simulink model "LF_AC29bus_HVDCdemo_V2_1"  (R2019b)
settings: Solver=FixedStepDiscrete  StartTime=0.0  StopTime=fix(6/Ts)*Ts  FixedStep=Ts  RelTol=1e-3
InitFcn:
  | Ts_avg=150e-6;
  | Ts=50e-6;
  | 
  | %Tc_stab = 1/60/5;
  | %Tc_stab = 2/60;
  | Tc_stab = Ts;
  | 
  | 
  | Ts_avg=150e-6;
  | 
  | Ts=50e-6;
  | 
  | % Rectifier AC side :
  | VLL_nom_R = 735e3; % V
  | Fnom_R = 60;           % Hz
  | 
  | % Inverter AC side :
  | VLL_nom_I = 735e3; % V
  | Fnom_I = 60;           % Hz
  | 
  | % DC :
  | Vdc_nom = 500e3;   % V
  | Idc_nom  = 2000;     % A
undefined symbols (not defined in the file): D1, D11, Delta, test_alpha
libraries: powerlib x223, powerlib_meascontrol x57, simulink x22, sps_avr x7
(part 3 of 10)

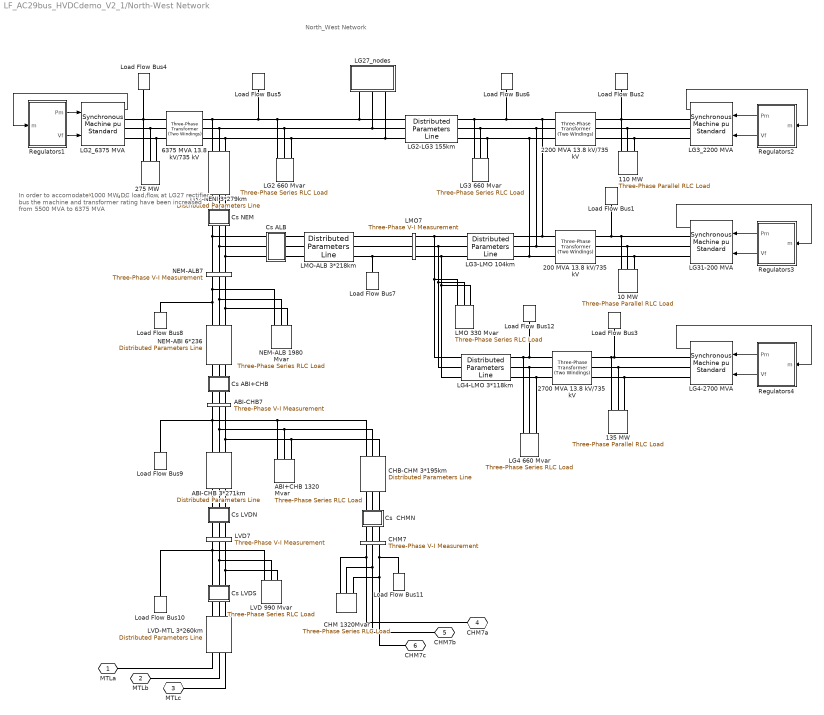
== system LF_AC29bus_HVDCdemo_V2_1/North-West Network ==
  note: North_West Network
  note: In order to accomodate 1000 MW
      | DC load flow at LG27 rectifier bus
      | the machine and transformer rating have been
      | increased from 5500 MVA to 6375 MVA
  10 MW : powerlib/Elements/Three-Phase Parallel RLC Load  LConnTagsString=A|B|C  Configuration=Y (grounded)  NominalVoltage=(13800)*1  Vabc=[1e3 1e3 1e3]  Vabcp=[1e3 1e3 1e3]  NominalFrequency=60  UnbalancedPower=off  ActivePower=10000000  InductivePower=0  CapacitivePower=0  Pabc=[10e3 9e3 11e3]  QLabc=[100 90 110]  QCabc=[100 90 110]  Pabcp=[10e3 9e3 11e3]  QLabcp=[100 90 110]  QCabcp=[100 90 110]  Measurements=None  LoadType=constant PQ
      settings: SourceProductName=Simscape Electrical
  110 MW : powerlib/Elements/Three-Phase Parallel RLC Load  LConnTagsString=A|B|C  Configuration=Y (grounded)  NominalVoltage=(13800)*1  Vabc=[1e3 1e3 1e3]  Vabcp=[1e3 1e3 1e3]  NominalFrequency=60  UnbalancedPower=off  ActivePower=110000000  InductivePower=0  CapacitivePower=0  Pabc=[10e3 9e3 11e3]  QLabc=[100 90 110]  QCabc=[100 90 110]  Pabcp=[10e3 9e3 11e3]  QLabcp=[100 90 110]  QCabcp=[100 90 110]  Measurements=None  LoadType=constant PQ
      settings: SourceProductName=Simscape Electrical
  135 MW : powerlib/Elements/Three-Phase Parallel RLC Load  LConnTagsString=A|B|C  Configuration=Y (grounded)  NominalVoltage=(13800)*1  Vabc=[1e3 1e3 1e3]  Vabcp=[1e3 1e3 1e3]  NominalFrequency=60  UnbalancedPower=off  ActivePower=135000000  InductivePower=0  CapacitivePower=0  Pabc=[10e3 9e3 11e3]  QLabc=[100 90 110]  QCabc=[100 90 110]  Pabcp=[10e3 9e3 11e3]  QLabcp=[100 90 110]  QCabcp=[100 90 110]  Measurements=None  LoadType=constant PQ
      settings: SourceProductName=Simscape Electrical
  200 MVA 13.8 kV/735 kV : powerlib/Elements/Three-Phase Transformer (Two Windings)  Winding1Connection=Delta (D1)  Winding2Connection=Yg  CoreType=Three single-phase transformers  SetSaturation=off  Hysteresis=off  DataFile='basic_model'  SetInitialFlux=off  Measurements=None  UNITS=pu  NominalPower=[ 200e6 60 ]  Winding1="[ 13.8e3 0.002  0.0]"  Winding2=[ 735e3 0.002 0.12]  Rm=500  Lm=500  L0=0.5  Saturation="[ 0,0  ;  0.005,1.2  ;  1.0,1.4 ]"  InitialFluxes=[ 0.8 , -0.8 , 0.7 ]  BreakLoop=off  DiscreteSolver=Trapezoidal iterative  DataType=off  TransfoNumber=0
      settings: SourceProductName=Simscape Electrical
  2200 MVA 13.8 kV/735 kV : powerlib/Elements/Three-Phase Transformer (Two Windings)  Winding1Connection=Delta (D1)  Winding2Connection=Yg  CoreType=Three single-phase transformers  SetSaturation=on  Hysteresis=off  DataFile='basic_model'  SetInitialFlux=off  Measurements=None  UNITS=pu  NominalPower=[ 2200e6 60 ]  Winding1="[ 13.8e3 0.002  0.0]"  Winding2=[ 735e3 0.002 0.12]  Rm=500  Lm=500  L0=0.5  Saturation="[ 0,0  ;  0.005,1.2  ;  1.0,1.4 ]"  InitialFluxes=[-0.877661878677196 -0.0593483795260228 0.937010258203213]  BreakLoop=off  DiscreteSolver=Trapezoidal iterative  DataType=off  TransfoNumber=0
      settings: SourceProductName=Simscape Electrical
  2700 MVA 13.8 kV/735 kV : powerlib/Elements/Three-Phase Transformer (Two Windings)  Winding1Connection=Delta (D1)  Winding2Connection=Yg  CoreType=Three single-phase transformers  SetSaturation=off  Hysteresis=off  DataFile='basic_model'  SetInitialFlux=off  Measurements=None  UNITS=pu  NominalPower=[ 2700e6 60 ]  Winding1="[ 13.8e3 0.002  0.0]"  Winding2=[ 735e3 0.002 0.12]  Rm=500  Lm=500  L0=0.5  Saturation="[ 0,0  ;  0.005,1.2  ;  1.0,1.4 ]"  InitialFluxes=[ 0.8 , -0.8 , 0.7 ]  BreakLoop=off  DiscreteSolver=Trapezoidal iterative  DataType=off  TransfoNumber=0
      settings: SourceProductName=Simscape Electrical
  275 MW : powerlib/Elements/Three-Phase Parallel RLC Load  LConnTagsString=A|B|C  Configuration=Y (grounded)  NominalVoltage=(13800)*1  Vabc=[1e3 1e3 1e3]  Vabcp=[1e3 1e3 1e3]  NominalFrequency=60  UnbalancedPower=off  ActivePower=275000000  InductivePower=0  CapacitivePower=0  Pabc=[10e3 9e3 11e3]  QLabc=[100 90 110]  QCabc=[100 90 110]  Pabcp=[10e3 9e3 11e3]  QLabcp=[100 90 110]  QCabcp=[100 90 110]  Measurements=None  LoadType=constant PQ
      settings: SourceProductName=Simscape Electrical
  6375 MVA 13.8 kV/735 kV : powerlib/Elements/Three-Phase Transformer (Two Windings)  Winding1Connection=Delta (D1)  Winding2Connection=Yg  CoreType=Three single-phase transformers  SetSaturation=off  Hysteresis=off  DataFile='basic_model'  SetInitialFlux=off  Measurements=None  UNITS=pu  NominalPower=[ 6375e6 60 ]  Winding1="[ 13.8e3 0.002  0.0]"  Winding2=[ 735e3 0.002 0.12]  Rm=500  Lm=500  L0=0.5  Saturation="[ 0,0  ;  0.005,1.2  ;  1.0,1.4 ]"  InitialFluxes=[-0.881083533460614 -0.0784579414635117 0.959541474924115]  BreakLoop=off  DiscreteSolver=Trapezoidal iterative  DataType=off  TransfoNumber=0
      settings: SourceProductName=Simscape Electrical
  ABI+CHB 1320 Mvar : powerlib/Elements/Three-Phase Series RLC Load  LConnTagsString=A|B|C  Configuration=Y (grounded)  NominalVoltage=735e3  Vabc=[1e3 1e3 1e3]  Vabcp=[1e3 1e3 1e3]  NominalFrequency=60  UnbalancedPower=off  ActivePower=4400000  InductivePower=1320e6  CapacitivePower=0  Pabc=[10e3 9e3 11e3]  QLabc=[100 90 110]  QCabc=[100 90 110]  Pabcp=[10e3 9e3 11e3]  QLabcp=[100 90 110]  QCabcp=[100 90 110]  Measurements=None  LoadType=constant Z
      settings: SourceProductName=Simscape Electrical
  ABI-CHB 3*271km : powerlib/Elements/Distributed Parameters Line  Phases=3  Frequency=60  Resistance="[0.01273  0.3864]/3"  Inductance="[0.9337e-3  4.1264e-3]/3"  Capacitance=[12.74e-9 7.751e-9]*3  Length=271  x1=[-0.00155 3.03044548903321e-09 4064.33950461954 -793349.443269264;-0.0015 2.84012543300991e-09 19017.0331579715 -793131.910667716;-0.00145 2.64879629394385e-09 33962.9701499944 -792632.582074898;-0.0014 2.45652605016711e-09 48896.8402604415 -791851.634899884;-0.00135 2.26338301438178e-09 63813.3375563722 -790789.346609484;-0.0013 2.06943580938881e-09 78707.1622773238 -789446.094629671;-0.00125 1.87475334370663e-09 93573.0227182919 -787822.356211476;-0.0012 1.67940478708828e-09 108405.637109847 -785918.708261429;-0.00115 1.48345954594577e-09 123199.735494723 -783735.827136581;-0.0011 1.28698723869025e-09 137950.061600208 -781274.488404202;-0.00105 1.09005767099697e-09 152651.374705672 -778535.566566224;-0.001 8.92740811003617e-10 167298.451504571 -775520.034748534;-0.00095 6.95106764451008e-10 181886.087960261 -772228.964355228;-0.0009 4.9722574977482e-10 196409.101154972 -768663.524687946;-0.00085 2.99168073157338e-10 210862.331131267 -764824.982530424;-0.0008 1.01004103547987e-10 225240.642725356 -760714.701698414;-0.00075 -9.71957523384118e-11 239538.927391596 -756334.142555123;-0.0007 -2.95361075036814e-10 253752.105017526 -751684.861492356;-0.00065 -4.93421457351652e-10 267875.125728814 -746768.510377537;-0.0006 -6.91306529372178e-10 281902.971683449 -741586.835966808;-0.00055 -8.88945983474555e-10 295830.65885456 -736141.679284413;-0.0005 -1.08626959930183e-09 309653.238801212 -730434.974968594;-0.00045 -1.28320726871286e-09 323365.800426569 -724468.75058422;-0.0004 -1.47968902069147e-09 336963.471722778 -718245.125902408;-0.00035 -1.67564504620674e-09 350441.421501976 -711766.312147371;-0.0003 -1.87100572301588e-09 363794.861112782 -705034.611210788;-0.00025 -2.06570164040064e-09 377019.046141687 -698052.414833947;-0.0002 -2.25966362382865e-09 390109.278098719 -690822.203757974;-0.00015 -2.45282275953077e-09 403060.906086794 -683346.546842438;-0.0001 -2.64511041898583e-09 415869.328454157 -675628.100152644;-5e-05 -2.83645828330403e-09 428529.994429332 -667669.606015948]  x2=[-0.00155 8.02624605987501e-09 -258398.582296341 -745155.265654966;-0.0015 7.70658744474234e-09 -244307.655094877 -749893.30711574;-0.00145 7.38419071578638e-09 -230129.926546857 -754364.915055201;-0.0014 7.05917041902979e-09 -215870.433931726 -758568.500732341;-0.00135 6.7316420326364e-09 -201534.243579312 -762502.570633184;-0.0013 6.40172192588232e-09 -187126.449069784 -766165.727001427;-0.00125 6.06952731781053e-09 -172652.169423925 -769556.668335055;-0.0012 5.73517623558349e-09 -158116.547284374 -772674.189848758;-0.00115 5.39878747254867e-09 -143524.747088463 -775517.183901988;-0.0011 5.06048054603181e-09 -128881.953233322 -778084.640392493;-0.00105 4.72037565487303e-09 -114193.368233883 -780375.647115209;-0.001 4.37859363672069e-09 -99464.2108744566 -782389.390086356;-0.00095 4.03525592509842e-09 -84699.7143545168 -784125.153832645;-0.0009 3.6904845062603e-09 -69905.1244293745 -785582.321645481;-0.00085 3.34440187584979e-09 -55085.697546384 -786760.375800079;-0.0008 2.99713099537756e-09 -40246.6989773522 -787658.897739409;-0.00075 2.64879524853386e-09 -25393.4009478132 -788277.568222902;-0.0007 2.29951839735091e-09 -10531.0807638311 -788616.167439882;-0.00065 1.9494245382308e-09 4334.98106300135 -788674.57508766;-0.0006 1.59863805785468e-09 19199.5026917037 -788452.770414276;-0.00055 1.24728358898871e-09 34057.2028285203 -787950.832225875;-0.0005 8.95485966202654e-10 48902.8026033394 -787168.938858705;-0.00045 5.43370181516771e-10 63731.02744525 -786107.368115756;-0.0004 1.91061339992716e-10 78536.6089565721 -784766.497168059;-0.00035 -1.61315384715677e-10 93314.2867846932 -783146.802420676;-0.0003 -5.13634794836002e-10 108058.810491047 -781248.859343439;-0.00025 -8.65771712959456e-10 122764.941416568 -779073.342266486;-0.0002 -1.21760102651577e-09 137427.454542963 -776621.024140676;-0.00015 -1.56899773222511e-09 152041.140349136 -773892.776262961;-0.0001 -1.91983698051116e-09 166600.806662105 -770889.567966821;-5e-05 -2.26999411985957e-09 181101.280501756 -767612.466277865]  x3=[-0.00155 7.187476204044e-11 -269.429023408063 -297.516890795202;-0.0015 7.16746615436663e-11 -263.773367075838 -302.542665626847;-0.00145 7.14490953809336e-11 -258.023993322279 -307.460948489986;-0.0014 7.11981436948253e-11 -252.182944872504 -312.269991942139;-0.00135 7.09218956472806e-11 -246.252297023214 -316.968087353065;-0.0013 7.06204493879154e-11 -240.234156905352 -321.553565511835;-0.00125 7.02939120191502e-11 -234.130662735444 -326.024797219895;-0.0012 6.99423995581575e-11 -227.943983055907 -330.380193869908;-0.00115 6.95660368956407e-11 -221.676315964573 -334.618208010183;-0.0011 6.91649577514617e-11 -215.329888333714 -338.737333894476;-0.00105 6.87393046271309e-11 -208.906955018849 -342.736108016974;-0.001 6.82892287551762e-11 -202.409798057601 -346.613109632272;-0.00095 6.78148900454121e-11 -195.840725858902 -350.366961260157;-0.0009 6.73164570281235e-11 -189.202072382823 -353.99632917502;-0.00085 6.6794106794188e-11 -182.496196311335 -357.499923879722;-0.0008 6.62480249321566e-11 -175.725480210274 -360.876500563748;-0.00075 6.56784054623145e-11 -168.892329682833 -364.12485954548;-0.0007 6.50854507677472e-11 -161.999172514856 -367.243846698439;-0.00065 6.44693715224342e-11 -155.048457812262 -370.23235386134;-0.0006 6.38303866163977e-11 -148.042655130889 -373.08931923182;-0.00055 6.31687230779324e-11 -140.984253599071 -375.813727743686;-0.0005 6.24846159929428e-11 -133.875761033263 -378.404611427566;-0.00045 6.17783084214188e-11 -126.719703047024 -380.861049754823;-0.0004 6.10500513110774e-11 -119.518622153684 -383.182169964618;-0.00035 6.03001034082022e-11 -112.275076862994 -385.367147373991;-0.0003 5.95287311657121e-11 -104.991640772106 -387.415205670873;-0.00025 5.87362086484918e-11 -97.6709016511821 -389.325617189904;-0.0002 5.79228174360182e-11 -90.3154605239728 -391.097703170967;-0.00015 5.70888465223159e-11 -82.927930743687 -392.730834000352;-0.0001 5.62345922132795e-11 -75.5109370644792 -394.22442943445;-5e-05 5.53603580213974e-11 -68.0671147088866 -395.577958805916]  x4=[-0.00155 -2.85924004000298e-12 -5537.83930789508 -16089.2052623055;-0.0015 -4.2812247881995e-12 -5233.59885671486 -16190.7265075691;-0.00145 -5.70168843761432e-12 -4927.49893278125 -16286.4952647987;-0.0014 -7.12012630427653e-12 -4619.64829193969 -16376.4775078107;-0.00135 -8.53603442396615e-12 -4310.156312057 -16460.6412663428;-0.0013 -9.94890973127026e-12 -3999.13295415996 -16538.9566374122;-0.00125 -1.13582502383198e-11 -3686.68872336665 -16611.3957959405;-0.0012 -1.27635552131433e-11 -3372.93462962453 -16677.9330046396;-0.00115 -1.41643253575747e-11 -3057.98214826913 -16738.5446231562;-0.0011 -1.55600629846517e-11 -2741.94318041739 -16793.2091164707;-0.00105 -1.69502721954413e-11 -2424.93001320974 -16841.9070625489;-0.001 -1.83344590552306e-11 -2107.05527991498 -16884.6211592426;-0.00095 -1.97121317690192e-11 -1788.43191991226 -16921.3362304365;-0.0009 -2.1082800856252e-11 -1469.17313856423 -16952.0392314407;-0.00085 -2.24459793247288e-11 -1149.39236699571 -16976.7192536251;-0.0008 -2.38011828436307e-11 -829.203221792158 -16995.3675282953;-0.00075 -2.51479299156004e-11 -508.719464632255 -17007.9774298081;-0.0007 -2.64857420478159e-11 -188.054961868896 -17014.5444779257;-0.00065 -2.78141439219968e-11 132.67635592697 -17015.066339407;-0.0006 -2.91326635632826e-11 453.360534445329 -17009.5428288371;-0.00055 -3.04408325079229e-11 773.883636124529 -16997.9759086931;-0.0005 -3.17381859697208e-11 1094.13178063275 -16980.3696886466;-0.00045 -3.30242630051688e-11 1413.99118532915 -16956.7304241038;-0.0004 -3.42986066772199e-11 1733.34820569029 -16927.0665139828;-0.00035 -3.55607642176355e-11 2052.0893756875 -16891.3884977295;-0.0003 -3.68102871878514e-11 2370.10144810078 -16849.7090515734;-0.00025 -3.80467316383059e-11 2687.27143475507 -16802.0429840231;-0.0002 -3.92696582661734e-11 3003.48664666436 -16748.4072306055;-0.00015 -4.04786325714459e-11 3318.63473406954 -16688.8208478484;-0.0001 -4.16732250113097e-11 3632.60372635577 -16623.3050065099;-5e-05 -4.28530111527589e-11 3945.28207183511 -16551.8829840563]  x5=0.00153261764655846  V1=ones(3,3)  V2=ones(3,3)  I1=ones(3,3)  I2=ones(3,3)  nHarmo=1  Measurements=None
      settings: AttributesFormatString=\n  SourceProductName=Simscape Electrical
  ABI-CHB7 : powerlib/Measurements/Three-Phase V-I Measurement  VoltageMeasurement=no  SetLabelV=on  LabelV=Vabc_ABI7  Vpu=on  VpuLL=off  CurrentMeasurement=no  SetLabelI=off  LabelI=A1  Ipu=off  Pbase=100e6  Vbase=500e3  OutputType=Magnitude  PhasorSimulation=off  PSBequivalent=0
      settings: SourceProductName=Simscape Electrical
  CHB-CHM 3*195km : powerlib/Elements/Distributed Parameters Line  Phases=3  Frequency=60  Resistance="[0.01273  0.3864]/3"  Inductance="[0.9337e-3  4.1264e-3]/3"  Capacitance=[12.74e-9 7.751e-9]*3  Length=195  x1=[-0.00115 1.48345954594577e-09 123199.735494723 -783735.827136581;-0.0011 1.28698723869025e-09 137950.061600208 -781274.488404202;-0.00105 1.09005767099697e-09 152651.374705672 -778535.566566224;-0.001 8.92740811003617e-10 167298.451504571 -775520.034748534;-0.00095 6.95106764451007e-10 181886.087960261 -772228.964355228;-0.0009 4.9722574977482e-10 196409.101154972 -768663.524687946;-0.00085 2.99168073157337e-10 210862.331131267 -764824.982530424;-0.0008 1.01004103547987e-10 225240.642725356 -760714.701698414;-0.00075 -9.71957523384118e-11 239538.927391596 -756334.142555123;-0.0007 -2.95361075036815e-10 253752.105017526 -751684.861492356;-0.00065 -4.93421457351653e-10 267875.125728814 -746768.510377537;-0.0006 -6.91306529372178e-10 281902.971683449 -741586.835966808;-0.00055 -8.88945983474555e-10 295830.65885456 -736141.679284413;-0.0005 -1.08626959930183e-09 309653.238801212 -730434.974968594;-0.00045 -1.28320726871286e-09 323365.800426569 -724468.75058422;-0.0004 -1.47968902069147e-09 336963.471722778 -718245.125902408;-0.00035 -1.67564504620674e-09 350441.421501976 -711766.312147371;-0.0003 -1.87100572301588e-09 363794.861112782 -705034.611210788;-0.00025 -2.06570164040064e-09 377019.046141687 -698052.414833947;-0.0002 -2.25966362382865e-09 390109.278098719 -690822.203757974;-0.00015 -2.45282275953077e-09 403060.906086794 -683346.546842438;-0.0001 -2.64511041898583e-09 415869.328454157 -675628.100152644;-5e-05 -2.83645828330403e-09 428529.994429332 -667669.606015948]  x2=[-0.00115 1.26948351703526e-09 19785.877107289 -777548.566694191;-0.0011 1.18361667340046e-09 34437.9555419689 -777037.519855601;-0.00105 1.09732929639752e-09 49077.7983350251 -776250.395286162;-0.001 1.01065204352065e-09 63700.2040200226 -775187.472647486;-0.00095 9.23615710785043e-10 78299.9773258478 -773849.129590925;-0.0009 8.36251221785304e-10 92871.9310225637 -772235.841623394;-0.00085 7.48589616708373e-10 107410.887764408 -770348.181938426;-0.0008 6.60662041305124e-10 121911.681929279 -768186.821212519;-0.00075 5.72499735824419e-10 136369.161454058 -765752.527366848;-0.0007 4.84134023913601e-10 150778.18966511 -763046.165294425;-0.00065 3.95596301489348e-10 165133.647103322 -760068.696552806;-0.0006 3.06918025582853e-10 179430.433343021 -756821.17902246;-0.00055 2.18130703163297e-10 193663.468804133 -753304.7665309;-0.0005 1.2926587994356e-10 207827.69655693 -749520.708442741;-0.00045 4.03551291721951e-11 221918.084118737 -745470.349215804;-0.0004 -4.85699595844092e-11 235929.625241945 -741155.127923435;-0.00035 -1.37477791665645e-10 249857.341692712 -736576.577743213;-0.0003 -2.26336778542119e-10 263696.285019701 -731736.325412215;-0.00025 -3.15115349038905e-10 277441.538312243 -726636.090649046;-0.0002 -4.03781960552638e-10 291088.217947293 -721277.685542834;-0.00015 -4.92305110258441e-10 304631.475324557 -715663.013909397;-0.0001 -5.80653346302739e-10 318066.498589178 -709794.070614833;-5e-05 -6.68795278977944e-10 331388.514341361 -703672.940866746]  x3=[-0.00115 -4.00870198362018e-11 363.641439526389 -4246.81013839968;-0.0011 -4.05597251460579e-11 443.622892755758 -4239.20169671289;-0.00105 -4.10180197786996e-11 523.446728883695 -4230.08708684871;-0.001 -4.14617409042261e-11 603.084586881312 -4219.46954718463;-0.00095 -4.18907308706343e-11 682.508171796869 -4207.35285008194;-0.0009 -4.23048372598317e-11 761.689264808829 -4193.74130054543;-0.00085 -4.27039129417903e-11 840.599733251876 -4178.63973469382;-0.0008 -4.30878161268203e-11 919.211540612314 -4162.05351804156;-0.00075 -4.34564104159482e-11 997.496756489306 -4143.98854359245;-0.0007 -4.38095648493782e-11 1075.42756651842 -4124.4512297459;-0.00065 -4.41471539530215e-11 1152.97628225392 -4103.44851801647;-0.0006 -4.44690577830773e-11 1230.11535100637 -4080.98787056765;-0.00055 -4.47751619686474e-11 1306.81736563194 -4057.07726756053;-0.0005 -4.50653577523722e-11 1383.05507427008 -4031.72520431849;-0.00045 -4.53395420290717e-11 1458.8013900259 -4004.94068830889;-0.0004 -4.55976173823778e-11 1534.0294005941 -3976.73323594273;-0.00035 -4.58394921193464e-11 1608.71237782074 -3947.11286919353;-0.0003 -4.60650803030351e-11 1682.8237871996 -3916.09011203654;-0.00025 -4.62743017830365e-11 1756.33729729984 -3883.67598670968;-0.0002 -4.64670822239549e-11 1829.22678912136 -3849.88200979732;-0.00015 -4.66433531318176e-11 1901.46636537478 -3814.72018813854;-0.0001 -4.68030518784104e-11 1973.03035968264 -3778.20301456116;-5e-05 -4.69461217235291e-11 2043.89334569852 -3740.34346344307]  x4=[-0.00115 6.12582094902268e-11 -985.140346861288 -13136.5681113659;-0.0011 6.07682415286824e-11 -737.361455949848 -13152.8029932245;-0.00105 6.02566829002781e-11 -489.320584024144 -13164.3647468082;-0.001 5.97237153593585e-11 -241.105858824892 -13171.2492642811;-0.00095 5.91695282667533e-11 7.19453013794555 -13173.4540996068;-0.0009 5.85943185224977e-11 255.492362918483 -13170.9784694179;-0.00085 5.79982904958747e-11 503.699420479033 -13163.8232532939;-0.0008 5.73816559528042e-11 751.727516033909 -13151.9909934492;-0.00075 5.67446339806033e-11 999.488526381779 -13135.4858938293;-0.0007 5.60874509101453e-11 1246.89442321541 -13114.3138186174;-0.00065 5.5410340235446e-11 1493.8573043977 -13088.4822901511;-0.0006 5.47135425307039e-11 1740.28942519292 -13058.0004862495;-0.00055 5.39973053648256e-11 1986.10322944197 -13022.8792369524;-0.0005 5.32618832134657e-11 2231.21138067066 -12983.1310206723;-0.00045 5.25075373686129e-11 2475.52679311997 -12938.7699597613;-0.0004 5.17345358457538e-11 2718.9626626872 -12889.8118154931;-0.00035 5.09431532886488e-11 2961.43249776703 -12836.2739824632;-0.0003 5.01336708717521e-11 3202.85014998162 -12778.1754824087;-0.00025 4.93063762003122e-11 3443.12984478868 -12715.5369574502;-0.0002 4.84615632081864e-11 3682.18621195674 -12648.3806627572;-0.00015 4.75995320534082e-11 3919.93431589687 -12576.7304586415;-0.0001 4.67205890115422e-11 4156.28968583978 -12500.6118020794;-5e-05 4.58250463668659e-11 4391.16834584798 -12420.0517376671]  x5=0.0011028060556417  V1=ones(3,3)  V2=ones(3,3)  I1=ones(3,3)  I2=ones(3,3)  nHarmo=1  Measurements=None
      settings: AttributesFormatString=\n  SourceProductName=Simscape Electrical
  CHM 1320Mvar : powerlib/Elements/Three-Phase Series RLC Load  LConnTagsString=A|B|C  Configuration=Y (grounded)  NominalVoltage=735e3  Vabc=[1e3 1e3 1e3]  Vabcp=[1e3 1e3 1e3]  NominalFrequency=60  UnbalancedPower=off  ActivePower=4400000  InductivePower=1320e6  CapacitivePower=0  Pabc=[10e3 9e3 11e3]  QLabc=[100 90 110]  QCabc=[100 90 110]  Pabcp=[10e3 9e3 11e3]  QLabcp=[100 90 110]  QCabcp=[100 90 110]  Measurements=None  LoadType=constant Z
      settings: SourceProductName=Simscape Electrical
  CHM7 : powerlib/Measurements/Three-Phase V-I Measurement  VoltageMeasurement=no  SetLabelV=on  LabelV=Vabc_CHM7  Vpu=on  VpuLL=off  CurrentMeasurement=no  SetLabelI=off  LabelI=A1  Ipu=off  Pbase=100e6  Vbase=735e3  OutputType=Magnitude  PhasorSimulation=off  PSBequivalent=0
      settings: SourceProductName=Simscape Electrical
  "Cs  CHMN " : Subsystem  mask{Xc=25/3}
      mask prompts: Xc "Condensator Reactance at  60Hz  (ohm):"
      mask help: Series Compensation
      mask init:
      | Cs=1/Xc/(2*pi*60);
      mask Display: disp('Cs')
  "Cs ABI+CHB " : Subsystem  mask{Xc=25/6}
      mask prompts: Xc "Condensator Reactance at  60Hz  (ohm):"
      mask help: Series Compensation
      mask init:
      | Cs=1/Xc/(2*pi*60);
      mask Display: disp('Cs')
  Cs ALB : Subsystem  mask{Xc=16/3}
      mask prompts: Xc "Reactance @ 60Hz du condensateur (ohm):"
      mask init:
      | Cs=1/Xc/(2*pi*60);
      mask Display: disp('Cs')
  "Cs LVDN " : Subsystem  mask{Xc=34/3}
      mask prompts: Xc "Condensator Reactance at  60Hz  (ohm):"
      mask help: Series Compensation
      mask init:
      | Cs=1/Xc/(2*pi*60);
      mask Display: disp('Cs')
  "Cs LVDS " : Subsystem  mask{Xc=34/3}
      mask prompts: Xc "Condensator Reactance at  60Hz  (ohm):"
      mask help: Series Compensation
      mask init:
      | Cs=1/Xc/(2*pi*60);
      mask Display: disp('Cs')
  "Cs NEM " : Subsystem  mask{Xc=16/3}
      mask prompts: Xc "Condensator Reactance at  60Hz  (ohm):"
      mask help: Series Compensation
      mask init:
      | Cs=1/Xc/(2*pi*60);
      mask Display: disp('Cs')
  LG2 660 Mvar : powerlib/Elements/Three-Phase Series RLC Load  LConnTagsString=A|B|C  Configuration=Y (grounded)  NominalVoltage=735e3  Vabc=[1e3 1e3 1e3]  Vabcp=[1e3 1e3 1e3]  NominalFrequency=60  UnbalancedPower=off  ActivePower=2200000  InductivePower=660e6  CapacitivePower=0  Pabc=[10e3 9e3 11e3]  QLabc=[100 90 110]  QCabc=[100 90 110]  Pabcp=[10e3 9e3 11e3]  QLabcp=[100 90 110]  QCabcp=[100 90 110]  Measurements=None  LoadType=constant Z
      settings: SourceProductName=Simscape Electrical
  LG2-LG3 155km : powerlib/Elements/Distributed Parameters Line  Phases=3  Frequency=60  Resistance="[0.01273  0.3864]"  Inductance="[0.9337e-3  4.1264e-3]"  Capacitance=[12.74e-9 7.751e-9]  Length=155  x1=[-0.0009 -1.73143034287158e-10 492501.296214061 -608754.179016124;-0.00085 -1.63865742472657e-10 503887.883804565 -599363.16237439;-0.0008 -1.54530229940123e-10 515095.442429276 -589759.194855004;-0.00075 -1.45139813552704e-10 526119.990095978 -579945.688701893;-0.0007 -1.35697829680631e-10 536957.609835383 -569926.130607067;-0.00065 -1.26207633015813e-10 547604.451092799 -559704.080471806;-0.0006 -1.16672595379938e-10 558056.731096226 -549283.170141851;-0.00055 -1.07096104526474e-10 568310.736200347 -538667.102117021;-0.0005 -9.74815629370227e-11 578362.823205975 -527859.648235736;-0.00045 -8.78323866124299e-11 588209.420654461 -516864.648334899;-0.0004 -7.8152003859098e-11 597847.030096616 -505686.00888562;-0.00035 -6.84438540709249e-11 607272.227335698 -494327.701605268;-0.0003 -5.87113865073038e-11 616481.663644005 -482793.762046336;-0.00025 -4.8958059067618e-11 625472.06695267 -471088.288162627;-0.0002 -3.9187337062665e-11 634240.243014206 -459215.438853277;-0.00015 -2.94026919834487e-11 642783.076537409 -447179.432485111;-0.0001 -1.96076002677751e-11 651097.532294205 -434984.545393881;-5e-05 -9.8055420650903e-12 659180.656198055 -422635.110364902]  x2=[-0.0009 -9.81346297235517e-10 481334.701264328 -598845.769358962;-0.00085 -9.48542840900518e-10 492536.517036616 -589666.993050645;-0.0008 -9.15402371810746e-10 503563.336929672 -580278.710867466;-0.00075 -8.81936664617066e-10 514411.243166893 -570684.258421382;-0.0007 -8.48157609525893e-10 525076.381538847 -560887.044575661;-0.00065 -8.14077208074658e-10 535554.962772653 -550890.550233732;-0.0006 -7.79707568867718e-10 545843.263878294 -540698.327102436;-0.00055 -7.4506090327423e-10 555937.629471377 -530313.996430119;-0.0005 -7.10149521089504e-10 565834.473071871 -519741.247720023;-0.00045 -6.74985826161395e-10 575530.27837837 -508983.837419421;-0.0004 -6.39582311983277e-10 585021.600517416 -498045.587584971;-0.00035 -6.03951557255156e-10 594305.067267448 -486930.384524754;-0.0003 -5.6810622141453e-10 603377.380256934 -475642.177417493;-0.00025 -5.3205904013854e-10 612235.316136267 -464184.976909421;-0.0002 -4.95822820819051e-10 620875.727723007 -452562.853689326;-0.00015 -4.59410438012244e-10 629295.545120061 -440779.937042245;-0.0001 -4.22834828864348e-10 637491.776806398 -428840.41338236;-5e-05 -3.86108988515134e-10 645461.510699929 -416748.524765573]  x3=[-0.0009 -4.99339044175808e-12 1757.33685624461 -2208.05664870762;-0.00085 -5.00391151599104e-12 1798.64327683998 -2174.54131821874;-0.0008 -5.01265472428907e-12 1839.31064804355 -2140.25338355384;-0.00075 -5.01961696023192e-12 1879.32452093196 -2105.20502705283;-0.0007 -5.02479575017029e-12 1918.67067876672 -2069.40870122989;-0.00065 -5.02818925410479e-12 1957.33514204528 -2032.87712434913;-0.0006 -5.02979626633962e-12 1995.30417346795 -1995.62327590588;-0.00055 -5.02961621591099e-12 2032.56428281867 -1957.66039201509;-0.0005 -5.02764916678995e-12 2069.102231758 -1919.00196070866;-0.00045 -5.0238958178597e-12 2104.90503852666 -1879.66171714313;-0.0004 -5.01835750266724e-12 2139.95998255788 -1839.65363871974;-0.00035 -5.01103618894958e-12 2174.25460899698 -1798.99194011824;-0.0003 -5.00193447793463e-12 2207.77673312646 -1757.69106824652;-0.00025 -4.99105560341697e-12 2240.51444469526 -1715.76569710771;-0.0002 -4.97840343060891e-12 2272.45611215033 -1673.23072258655;-0.00015 -4.96398245476722e-12 2303.59038676932 -1630.10125715693;-0.0001 -4.94779779959593e-12 2333.90620669271 -1586.39262451256;-5e-05 -4.92985521542598e-12 2363.39280085403 -1542.1203541225]  x4=[-0.0009 3.66787403448836e-12 1370.82791492966 -2590.65339627375;-0.00085 3.73088013352556e-12 1419.41409254251 -2564.35529770361;-0.0008 3.79256066861634e-12 1467.49595908698 -2537.14609590667;-0.00075 3.85289372496029e-12 1515.05643130484 -2509.03545818278;-0.0007 3.91185786650977e-12 1562.07861118679 -2480.03337210767;-0.00065 3.96943214358605e-12 1608.54579197619 -2450.15014198442;-0.0006 4.02559610032264e-12 1654.441464105 -2419.3963851824;-0.00055 4.08032978193313e-12 1699.74932105942 -2387.78302836497;-0.0005 4.13361374180108e-12 1744.45326517362 -2355.32130360726;-0.00045 4.18542904838925e-12 1788.53741334914 -2322.02274440553;-0.0004 4.23575729196594e-12 1831.98610269802 -2287.8991815793;-0.00035 4.28458059114585e-12 1874.78389610782 -2252.96273906795;-0.0003 4.33188159924327e-12 1916.91558772635 -2217.22582962316;-0.00025 4.37764351043524e-12 1958.36620836418 -2180.70115039869;-0.0002 4.42185006573262e-12 1999.12103081317 -2143.40167843914;-0.00015 4.46448555875681e-12 2039.16557507896 -2105.34066606931;-0.0001 4.50553484132014e-12 2078.48561352565 -2066.53163618565;-5e-05 4.54498332880799e-12 2117.06717593081 -2026.98837745169]  x5=0.000876589428843401  V1=ones(3,3)  V2=ones(3,3)  I1=ones(3,3)  I2=ones(3,3)  nHarmo=1  Measurements=None
      settings: AttributesFormatString=\n  SourceProductName=Simscape Electrical
  LG2-NENI 3*279km : powerlib/Elements/Distributed Parameters Line  Phases=3  Frequency=60  Resistance="[0.01273  0.3864]/3"  Inductance="[0.9337e-3  4.1264e-3]/3"  Capacitance=[12.74e-9 7.751e-9]*3  Length=279  x1=[-0.0016 -2.95110875322739e-10 0 0;-0.00155 -2.86983266050322e-10 0 0;-0.0015 -2.78753692989982e-10 0 0;-0.00145 -2.70425080069841e-10 0 0;-0.0014 -2.62000386406412e-10 0 0;-0.00135 -2.53482605253239e-10 0 0;-0.0013 -2.44874762937407e-10 0 0;-0.00125 -2.36179917784303e-10 0 0;-0.0012 -2.27401159031009e-10 0 0;-0.00115 -2.18541605728709e-10 0 0;-0.0011 -2.09604405634505e-10 0 0;-0.00105 -2.00592734093035e-10 0 0;-0.001 -1.91509792908287e-10 469207.278707835 -626884.09017855;-0.00095 -1.82358809206016e-10 480939.725258115 -617928.908196707;-0.0009 -1.73143034287158e-10 492501.296214061 -608754.179016124;-0.00085 -1.63865742472657e-10 503887.883804565 -599363.16237439;-0.0008 -1.54530229940123e-10 515095.442429276 -589759.194855004;-0.00075 -1.45139813552704e-10 526119.990095978 -579945.688701893;-0.0007 -1.35697829680631e-10 536957.609835383 -569926.130607067;-0.00065 -1.26207633015813e-10 547604.451092799 -559704.080471806;-0.0006 -1.16672595379938e-10 558056.731096226 -549283.170141851;-0.00055 -1.07096104526474e-10 568310.736200347 -538667.102117021;-0.0005 -9.74815629370227e-11 578362.823205975 -527859.648235736;-0.00045 -8.78323866124299e-11 588209.420654461 -516864.648334899;-0.0004 -7.8152003859098e-11 597847.030096616 -505686.00888562;-0.00035 -6.84438540709249e-11 607272.227335698 -494327.701605268;-0.0003 -5.87113865073038e-11 616481.663644005 -482793.762046336;-0.00025 -4.8958059067618e-11 625472.06695267 -471088.288162627;-0.0002 -3.9187337062665e-11 634240.243014206 -459215.438853277;-0.00015 -2.94026919834487e-11 642783.076537409 -447179.432485111;-0.0001 -1.96076002677751e-11 651097.532294205 -434984.545393881;-5e-05 -9.8055420650903e-12 659180.656198055 -422635.110364902]  x2=[-0.0016 2.61186761341134e-09 0 0;-0.00155 2.48578125998528e-09 0 0;-0.0015 2.35881172031388e-09 0 0;-0.00145 2.23100410607001e-09 0 0;-0.0014 2.10240382669045e-09 0 0;-0.00135 1.97305657324211e-09 0 0;-0.0013 1.84300830218824e-09 0 0;-0.00125 1.7123052190603e-09 0 0;-0.0012 1.58099376204137e-09 0 0;-0.00115 1.44912058546688e-09 0 0;-0.0011 1.31673254324853e-09 0 0;-0.00105 1.18387667222734e-09 0 0;-0.001 1.05060017546168e-09 247905.466622601 -744639.522916616;-0.00095 9.16950405456235e-10 261896.734704826 -739834.622582827;-0.0009 7.82974847337897e-10 275794.952124262 -734766.862530445;-0.00085 6.48721101984527e-10 289595.180910439 -729438.043310484;-0.0008 5.14236869112584e-10 303292.51790778 -723850.058227041;-0.00075 3.79569930329645e-10 316882.096517672 -718004.892664607;-0.0007 2.44768132157827e-10 330359.088427542 -711904.623382675;-0.00065 1.09879369034145e-10 343718.705326338 -705551.417777872;-0.0006 -2.50484337061505e-11 356956.200605788 -698947.5331139;-0.00055 -1.59967336857222e-10 370066.871046853 -692095.315719533;-0.0005 -2.94829404375211e-10 383046.058490751 -684997.200154984;-0.00045 -4.2958672040969e-10 395889.151493987 -677655.708346916;-0.0004 -5.64191406327936e-10 408591.58696677 -670073.44869241;-0.00035 -6.98595637725978e-10 421148.85179426 -662253.115132216;-0.0003 -8.32751661420381e-10 433556.484440058 -654197.486193613;-0.00025 -9.66611812414727e-10 445810.076531365 -645909.424003204;-0.0002 -1.10012853083476e-09 457905.274425258 -637391.87327002;-0.00015 -1.23325437882618e-09 469837.780755517 -628647.86023928;-0.0001 -1.36594205740908e-09 481603.355959462 -619680.491617178;-5e-05 -1.49814442328308e-09 493197.819784246 -610492.953467087]  x3=[-0.0016 4.83571502574089e-11 0 0;-0.00155 4.84725302681818e-11 0 0;-0.0015 4.85706882197581e-11 0 0;-0.00145 4.86515892370849e-11 0 0;-0.0014 4.87152045764161e-11 0 0;-0.00135 4.87615116355245e-11 0 0;-0.0013 4.87904939617325e-11 0 0;-0.00125 4.88021412577576e-11 0 0;-0.0012 4.8796449385371e-11 0 0;-0.00115 4.87734203668678e-11 0 0;-0.0011 4.87330623843486e-11 0 0;-0.00105 4.86753897768125e-11 0 0;-0.001 4.86004230350623e-11 -7.33523479552503 -1096.81827708524;-0.00095 4.85081887944245e-11 13.3397518919095 -1096.76170171712;-0.0009 4.83987198252854e-11 34.0099990290158 -1096.31545213874;-0.00085 4.82720550214486e-11 54.6681625754095 -1095.47968690046;-0.0008 4.81282393863158e-11 75.3069027839492 -1094.25470294567;-0.00075 4.79673240168973e-11 95.9188868085124 -1092.64093550535;-0.0007 4.77893660856577e-11 116.496791309322 -1090.63895794339;-0.00065 4.75944288202025e-11 137.033305054892 -1088.24948155287;-0.0006 4.73825814808141e-11 157.521131519676 -1085.47335530339;-0.00055 4.71538993358432e-11 177.952991476487 -1082.31156553937;-0.0005 4.69084636349672e-11 198.321625582771 -1078.76523562968;-0.00045 4.66463615803218e-11 218.619796959817 -1074.83562556843;-0.0004 4.63676862955192e-11 238.840293763987 -1070.52413152737;-0.00035 4.60725367925609e-11 258.975931749049 -1065.83228535981;-0.0003 4.57610179366601e-11 279.019556818705 -1060.76175405635;-0.00025 4.54332404089828e-11 298.964047568408 -1055.31433915262;-0.0002 4.5089320667324e-11 318.802317815562 -1049.49197608918;-0.00015 4.47293809047302e-11 338.527319117212 -1043.29673352393;-0.0001 4.43535490060852e-11 358.132043274316 -1036.73081259703;-5e-05 4.3961958502673e-11 377.609524821734 -1029.79654614893]  x4=[-0.0016 -3.41176914926163e-11 0 0;-0.00155 -3.48059164992901e-11 0 0;-0.0015 -3.54817751295642e-11 0 0;-0.00145 -3.61450272540854e-11 0 0;-0.0014 -3.6795437222532e-11 0 0;-0.00135 -3.74327739473393e-11 0 0;-0.0013 -3.80568109858037e-11 0 0;-0.00125 -3.86673266205368e-11 0 0;-0.0012 -3.92641039382407e-11 0 0;-0.00115 -3.9846930906776e-11 0 0;-0.0011 -4.0415600450496e-11 0 0;-0.00105 -4.09699105238196e-11 0 0;-0.001 -4.15096641830171e-11 5106.27611219788 -15399.3340454631;-0.00095 -4.20346696561835e-11 5395.62239341556 -15300.3532233518;-0.0009 -4.25447404113742e-11 5683.05163568875 -15195.9362585947;-0.00085 -4.30396952228785e-11 5968.4617167763 -15086.1202500422;-0.0008 -4.35193582356087e-11 6251.75123183542 -14970.9442147991;-0.00075 -4.39835590275803e-11 6532.81952945031 -14850.4490743625;-0.0007 -4.44321326704624e-11 6811.56674739319 -14724.6776400818;-0.00065 -4.48649197881754e-11 7087.8938481048 -14593.674597949;-0.0006 -4.52817666135174e-11 7361.70265388201 -14457.486492721;-0.00055 -4.5682525042796e-11 7632.89588175992 -14316.1617113832;-0.0005 -4.60670526884497e-11 7901.37717807598 -14169.7504659574;-0.00045 -4.64352129296369e-11 8167.051152704 -14018.304775662;-0.0004 -4.67868749607769e-11 8429.82341294584 -13861.8784484297;-0.00035 -4.71219138380246e-11 8689.60059706867 -13700.5270617895;-0.0003 -4.74402105236622e-11 8946.29040747591 -13534.307943121;-0.00025 -4.77416519283929e-11 9199.8016435002 -13363.2801492855;-0.0002 -4.80261309515209e-11 9450.0442338065 -13187.5044456438;-0.00015 -4.8293546519004e-11 9696.92926839401 -13007.0432844664;-0.0001 -4.85438036193643e-11 9940.36903018555 -12821.9607827447;-5e-05 -4.87768133374456e-11 10180.2770261929 -12632.3226994101]  x5=0.00157786097191812  V1=ones(3,3)  V2=ones(3,3)  I1=ones(3,3)  I2=ones(3,3)  nHarmo=1  Measurements=None
      settings: AttributesFormatString=\n  SourceProductName=Simscape Electrical
  LG27_nodes : Subsystem
  LG2_6375 MVA : powerlib/Machines/Synchronous Machine pu Standard  PresetModel=No  MechanicalLoad=Mechanical power Pm  ShowDetailedParameters=on  RotorType=Salient-pole  Units=per unit standard parameters  MeasurementBus=off  NominalParameters="[6375E6  13800   60 ]"  Reactances1=[ 31 32 33 34 35 36 37 ]  Reactances2=[ 1.305, 0.296, 0.252, 0.474, 0.243, 0.18 ]  dAxisTimeConstants=Short-circuit  qAxisTimeConstants=Open-circuit  TimeConstants1=[]  TimeConstants2=[]  TimeConstants3=[]  TimeConstants4=[]  TimeConstants5=[ 1.01, 0.053, 0.1 ]  TimeConstants6=[]  TimeConstants7=[]  TimeConstants8=[]  StatorResistance=2.8544e-3  Mechanical="[ 4.1  0  32]"  PolePairs=32  InitialConditions=[0 -65.2822 0.95354 0.95354 0.95354 2.75188 -117.248 122.752 1.37637]  SetSaturation=off  Saturation=[0.6404,0.7127,0.8441,0.9214,0.9956,1.082,1.19,1.316,1.457;0.7,0.7698,0.8872,0.9466,0.9969,1.046,1.1,1.151,1.201]  LoadFlowParameters=[2 4000000000 0 0 0]  TsPowergui=0  TsBlock=-1  IterativeModel=Trapezoidal non iterative  IterativeDiscreteModel=Trapezoidal non iterative  BusType=swing  Pref=0  Qref=0  Qmin=-Inf  Qmax=Inf  PLF=0  QLF=0
      settings: AttributesFormatString=\n\n  SourceProductName=Simscape Electrical
  LG3 660 Mvar : powerlib/Elements/Three-Phase Series RLC Load  LConnTagsString=A|B|C  Configuration=Y (grounded)  NominalVoltage=735e3  Vabc=[1e3 1e3 1e3]  Vabcp=[1e3 1e3 1e3]  NominalFrequency=60  UnbalancedPower=off  ActivePower=2200000  InductivePower=660e6  CapacitivePower=0  Pabc=[10e3 9e3 11e3]  QLabc=[100 90 110]  QCabc=[100 90 110]  Pabcp=[10e3 9e3 11e3]  QLabcp=[100 90 110]  QCabcp=[100 90 110]  Measurements=None  LoadType=constant Z
      settings: SourceProductName=Simscape Electrical
  LG3-LMO 104km : powerlib/Elements/Distributed Parameters Line  Phases=3  Frequency=60  Resistance="[0.01273  0.3864]"  Inductance="[0.9337e-3  4.1264e-3]"  Capacitance=[12.74e-9 7.751e-9]  Length=104  x1=[-0.0006 -7.79707568867718e-10 545843.263878294 -540698.327102436;-0.00055 -7.4506090327423e-10 555937.629471377 -530313.996430119;-0.0005 -7.10149521089504e-10 565834.473071871 -519741.247720023;-0.00045 -6.74985826161395e-10 575530.27837837 -508983.837419421;-0.0004 -6.39582311983277e-10 585021.600517416 -498045.587584971;-0.00035 -6.03951557255156e-10 594305.067267448 -486930.384524754;-0.0003 -5.6810622141453e-10 603377.380256934 -475642.177417493;-0.00025 -5.3205904013854e-10 612235.316136267 -464184.976909421;-0.0002 -4.95822820819051e-10 620875.727723007 -452562.853689326;-0.00015 -4.59410438012244e-10 629295.545120061 -440779.937042245;-0.0001 -4.22834828864348e-10 637491.776806398 -428840.41338236;-5e-05 -3.86108988515134e-10 645461.510699929 -416748.524765573]  x2=[-0.0006 -1.22744945109194e-09 483273.708399804 -611077.959257191;-0.00055 -1.30770287503563e-09 494705.735797608 -601860.466006677;-0.0005 -1.38749167837461e-09 505961.996603083 -592429.134598422;-0.00045 -1.46678751252696e-09 517038.491520362 -582787.315939564;-0.0004 -1.54556220406039e-09 527931.285123544 -572938.435722364;-0.00035 -1.6237877647021e-09 538636.507254928 -562885.993207066;-0.0003 -1.70143640128287e-09 549150.354400067 -552633.559978629;-0.00025 -1.77848052561185e-09 559469.091039131 -542184.778677761;-0.0002 -1.85489276427853e-09 569589.050974127 -531543.361706707;-0.00015 -1.93064596837834e-09 579506.638631477 -520713.089910244;-0.0001 -2.0057132231586e-09 589218.330339511 -509697.811232373;-5e-05 -2.0800678575811e-09 598720.675580408 -498501.439349158]  x3=[-0.0006 3.34879175457913e-11 -108.768475726974 -487.353741531589;-0.00055 3.3290724057145e-11 -99.5631949763572 -489.317335083408;-0.0005 3.30817025327588e-11 -90.3225398966472 -491.107076516015;-0.00045 3.28609272369853e-11 -81.0497936485933 -492.722329942799;-0.0004 3.26284766102356e-11 -71.7482507947842 -494.162521471911;-0.00035 3.23844332411106e-11 -62.4212161291055 -495.427139410157;-0.0003 3.21288838370574e-11 -53.0720035025621 -496.515734444805;-0.00025 3.18619191935624e-11 -43.7039346458829 -497.427919803223;-0.0002 3.15836341618921e-11 -34.3203379893254 -498.163371390297;-0.00015 3.12941276153934e-11 -24.9245474801007 -498.721827903579;-0.0001 3.09935024143635e-11 -15.5199013978374 -499.10309092613;-5e-05 3.06818653695051e-11 -6.10974116850738 -499.307024997014]  x4=[-0.0006 -3.56256684434537e-11 3608.8611189274 -4008.34009759276;-0.00055 -3.55086226366989e-11 3683.77097861045 -3939.60669378086;-0.0005 -3.53789607853999e-11 3757.37201200552 -3869.47356646956;-0.00045 -3.52367289577948e-11 3829.63806901588 -3797.96563362506;-0.0004 -3.50819776881749e-11 3900.5434738556 -3725.10830167538;-0.00035 -3.49147619589294e-11 3970.06303417196 -3650.92745648367;-0.0003 -3.47351411810106e-11 4038.1720499962 -3575.44945415099;-0.00025 -3.45431791728257e-11 4104.84632251931 -3498.70111165217;-0.0002 -3.43389441375621e-11 4170.06216268973 -3420.70969730786;-0.00015 -3.41225086389554e-11 4233.79639963 -3341.50292109621;-0.0001 -3.38939495755076e-11 4296.0263888692 -3261.10892480766;-5e-05 -3.36533481531657e-11 4356.73002038847 -3179.55627204627]  x5=0.000588163229675572  V1=ones(3,3)  V2=ones(3,3)  I1=ones(3,3)  I2=ones(3,3)  nHarmo=1  Measurements=None
      settings: AttributesFormatString=\n  SourceProductName=Simscape Electrical
  LG31-200 MVA : powerlib/Machines/Synchronous Machine pu Standard  PresetModel=No  MechanicalLoad=Mechanical power Pm  ShowDetailedParameters=on  RotorType=Salient-pole  Units=per unit standard parameters  MeasurementBus=off  NominalParameters="[200E6  13800   60 ]"  Reactances1=[ 31 32 33 34 35 36 37 ]  Reactances2=[ 1.305, 0.296, 0.252, 0.474, 0.243, 0.18 ]  dAxisTimeConstants=Short-circuit  qAxisTimeConstants=Open-circuit  TimeConstants1=[]  TimeConstants2=[]  TimeConstants3=[]  TimeConstants4=[]  TimeConstants5=[ 1.01, 0.053, 0.1 ]  TimeConstants6=[]  TimeConstants7=[]  TimeConstants8=[]  StatorResistance=2.8544e-3  Mechanical="[ 3.2  0  32]"  PolePairs=32  InitialConditions=[0 -66.4936 0.900145 0.900145 0.900145 -0.412002 -120.412 119.588 1.39985]  SetSaturation=off  Saturation=[0.6404,0.7127,0.8441,0.9214,0.9956,1.082,1.19,1.316,1.457;0.7,0.7698,0.8872,0.9466,0.9969,1.046,1.1,1.151,1.201]  LoadFlowParameters=[1 180000000 0 0 0]  TsPowergui=0  TsBlock=-1  IterativeModel=Trapezoidal non iterative  IterativeDiscreteModel=Trapezoidal non iterative  BusType=PV  Pref=180000000  Qref=0  Qmin=-Inf  Qmax=Inf  PLF=0  QLF=0
      settings: AttributesFormatString=\n\n  SourceProductName=Simscape Electrical
  LG3_2200 MVA : powerlib/Machines/Synchronous Machine pu Standard  PresetModel=No  MechanicalLoad=Mechanical power Pm  ShowDetailedParameters=on  RotorType=Salient-pole  Units=per unit standard parameters  MeasurementBus=off  NominalParameters="[2200E6  13800   60 ]"  Reactances1=[ 31 32 33 34 35 36 37 ]  Reactances2=[ 1.305, 0.296, 0.252, 0.474, 0.243, 0.18 ]  dAxisTimeConstants=Short-circuit  qAxisTimeConstants=Open-circuit  TimeConstants1=[]  TimeConstants2=[]  TimeConstants3=[]  TimeConstants4=[]  TimeConstants5=[ 1.01, 0.053, 0.1 ]  TimeConstants6=[]  TimeConstants7=[]  TimeConstants8=[]  StatorResistance=2.8544e-3  Mechanical="[ 3.2  0  32]"  PolePairs=32  InitialConditions=[0 -68.8789 0.818231 0.818231 0.818231 -0.573883 -120.574 119.426 1.33004]  SetSaturation=off  Saturation=[0.6404,0.7127,0.8441,0.9214,0.9956,1.082,1.19,1.316,1.457;0.7,0.7698,0.8872,0.9466,0.9969,1.046,1.1,1.151,1.201]  LoadFlowParameters=[1 1800000000 0 0 0]  TsPowergui=0  TsBlock=-1  IterativeModel=Trapezoidal non iterative  IterativeDiscreteModel=Trapezoidal non iterative  BusType=PV  Pref=1800000000  Qref=0  Qmin=-Inf  Qmax=Inf  PLF=0  QLF=0
      settings: AttributesFormatString=\n\n  SourceProductName=Simscape Electrical
  LG4 660 Mvar : powerlib/Elements/Three-Phase Series RLC Load  LConnTagsString=A|B|C  Configuration=Y (grounded)  NominalVoltage=735e3  Vabc=[1e3 1e3 1e3]  Vabcp=[1e3 1e3 1e3]  NominalFrequency=60  UnbalancedPower=off  ActivePower=2200000  InductivePower=660e6  CapacitivePower=0  Pabc=[10e3 9e3 11e3]  QLabc=[100 90 110]  QCabc=[100 90 110]  Pabcp=[10e3 9e3 11e3]  QLabcp=[100 90 110]  QCabcp=[100 90 110]  Measurements=None  LoadType=constant Z
      settings: SourceProductName=Simscape Electrical
  LG4-2700 MVA : powerlib/Machines/Synchronous Machine pu Standard  PresetModel=No  MechanicalLoad=Mechanical power Pm  ShowDetailedParameters=on  RotorType=Salient-pole  Units=per unit standard parameters  MeasurementBus=off  NominalParameters="[2700E6  13800   60 ]"  Reactances1=[ 31 32 33 34 35 36 37 ]  Reactances2=[ 1.305, 0.296, 0.252, 0.474, 0.243, 0.18 ]  dAxisTimeConstants=Short-circuit  qAxisTimeConstants=Open-circuit  TimeConstants1=[]  TimeConstants2=[]  TimeConstants3=[]  TimeConstants4=[]  TimeConstants5=[ 1.01, 0.053, 0.1 ]  TimeConstants6=[]  TimeConstants7=[]  TimeConstants8=[]  StatorResistance=2.8544e-3  Mechanical="[ 3.7  0  32]"  PolePairs=32  InitialConditions=[0 -67.8071 0.929463 0.929463 0.929463 2.70815 -117.292 122.708 1.31716]  SetSaturation=off  Saturation=[0.6404,0.7127,0.8441,0.9214,0.9956,1.082,1.19,1.316,1.457;0.7,0.7698,0.8872,0.9466,0.9969,1.046,1.1,1.151,1.201]  LoadFlowParameters=[1 2500000000 0 0 0]  TsPowergui=0  TsBlock=-1  IterativeModel=Trapezoidal non iterative  IterativeDiscreteModel=Trapezoidal non iterative  BusType=PV  Pref=2500000000  Qref=0  Qmin=-Inf  Qmax=Inf  PLF=0  QLF=0
      settings: AttributesFormatString=\n\n  SourceProductName=Simscape Electrical
  LG4-LMO 3*118km : powerlib/Elements/Distributed Parameters Line  Phases=3  Frequency=60  Resistance="[0.01273  0.3864]/3"  Inductance="[0.9337e-3  4.1264e-3]/3"  Capacitance=[12.74e-9 7.751e-9]*3  Length=118  x1=[-0.0007 -1.11451881767954e-09 488418.907412292 -593939.677725633;-0.00065 -1.1627563412782e-09 499526.992280968 -584628.251976426;-0.0006 -1.21058074308541e-09 510457.597587843 -575109.110593068;-0.00055 -1.25797503131892e-09 521206.839740899 -565385.635681167;-0.0005 -1.3049223670138e-09 531770.899585583 -555461.281945058;-0.00045 -1.35140607000523e-09 542146.023761734 -545339.575460369;-0.0004 -1.39740962485486e-09 552328.526037136 -535024.112421217;-0.00035 -1.44291668671871e-09 562314.788617213 -524518.557862502;-0.0003 -1.48791108715438e-09 572101.263430423 -513826.644357736;-0.00025 -1.53237683986566e-09 581684.473388864 -502952.170692876;-0.0002 -1.57629814638232e-09 591061.013623669 -491899.000516635;-0.00015 -1.6196594016733e-09 600227.55269474 -480671.060967745;-0.0001 -1.66244519969107e-09 609180.833774393 -469272.341279666;-5e-05 -1.70464033884532e-09 617917.675804493 -457706.891363225]  x2=[-0.0007 -1.06566295097469e-09 459898.661812722 -628858.40869839;-0.00065 -1.14675992020292e-09 471669.976154571 -620078.3394185;-0.0006 -1.22744945109194e-09 483273.708399804 -611077.959257191;-0.00055 -1.30770287503563e-09 494705.735797608 -601860.466006677;-0.0005 -1.38749167837461e-09 505961.996603083 -592429.134598422;-0.00045 -1.46678751252696e-09 517038.491520362 -582787.315939564;-0.0004 -1.54556220406039e-09 527931.285123544 -572938.435722364;-0.00035 -1.6237877647021e-09 538636.507254928 -562885.993207066;-0.0003 -1.70143640128287e-09 549150.354400067 -552633.559978629;-0.00025 -1.77848052561185e-09 559469.091039131 -542184.778677761;-0.0002 -1.85489276427853e-09 569589.050974127 -531543.361706707;-0.00015 -1.93064596837834e-09 579506.638631477 -520713.089910244;-0.0001 -2.0057132231586e-09 589218.330339511 -509697.811232373;-5e-05 -2.0800678575811e-09 598720.675580408 -498501.439349158]  x3=[-0.0007 1.83521676419456e-11 2289.61299645148 -5000.41594159407;-0.00065 1.79604628581857e-11 2383.45629751133 -4956.37225355976;-0.0006 1.75623768074931e-11 2476.45276789778 -4910.56759006411;-0.00055 1.71580509279462e-11 2568.56936640771 -4863.01822528596;-0.0005 1.67476288746047e-11 2659.77336445231 -4813.7410532882;-0.00045 1.63312564684698e-11 2750.03235768535 -4762.7535820154;-0.0004 1.59090816446749e-11 2839.3142775163 -4710.07392707332;-0.00035 1.54812543999246e-11 2927.58740250418 -4655.72080529253;-0.0003 1.50479267392018e-11 3014.82036962801 -4599.71352807838;-0.00025 1.46092526217611e-11 3100.98218542992 -4542.07199454979;-0.0002 1.41653879064276e-11 3186.04223702705 -4482.81668446914;-0.00015 1.3716490296221e-11 3269.97030298808 -4421.96865096596;-0.0001 1.32627192823249e-11 3352.73656407081 -4359.54951305682;-5e-05 1.28042360874198e-11 3434.31161381677 -4295.5814479642]  x4=[-0.0007 -3.00041942768163e-11 7136.87128691293 -9299.28340320072;-0.00065 -3.03582000941956e-11 7310.8807733927 -9163.11266463541;-0.0006 -3.07014197876356e-11 7482.29273874531 -9023.68631577159;-0.00055 -3.10337314128135e-11 7651.04628111566 -8881.05389412713;-0.0005 -3.13550169009912e-11 7817.08144317369 -8735.26607632228;-0.00045 -3.16651621009646e-11 7980.33923341691 -8586.3746600745;-0.0004 -3.19640568196209e-11 8140.76164712983 -8434.43254579504;-0.00035 -3.22515948610899e-11 8298.29168699273 -8279.4937177936;-0.0003 -3.25276740644745e-11 8452.87338333252 -8121.61322509802;-0.00025 -3.27921963401483e-11 8604.45181400858 -7960.84716189558;-0.0002 -3.30450677046064e-11 8752.97312392623 -7797.25264760303;-0.00015 -3.3286198313857e-11 8898.38454417127 -7630.88780657233;-0.0001 -3.35155024953429e-11 9040.63441075846 -7461.81174743933;-5e-05 -3.37328987783802e-11 9179.67218298757 -7290.08454212275]  x5=0.000667339049054976  V1=ones(3,3)  V2=ones(3,3)  I1=ones(3,3)  I2=ones(3,3)  nHarmo=1  Measurements=None
      settings: AttributesFormatString=\n  SourceProductName=Simscape Electrical
  LMO 330 Mvar : powerlib/Elements/Three-Phase Series RLC Load  LConnTagsString=A|B|C  Configuration=Y (grounded)  NominalVoltage=735e3  Vabc=[1e3 1e3 1e3]  Vabcp=[1e3 1e3 1e3]  NominalFrequency=60  UnbalancedPower=off  ActivePower=1100000  InductivePower=330e6  CapacitivePower=0  Pabc=[10e3 9e3 11e3]  QLabc=[100 90 110]  QCabc=[100 90 110]  Pabcp=[10e3 9e3 11e3]  QLabcp=[100 90 110]  QCabcp=[100 90 110]  Measurements=None  LoadType=constant Z
      settings: SourceProductName=Simscape Electrical
  LMO-ALB 3*218km : powerlib/Elements/Distributed Parameters Line  Phases=3  Frequency=60  Resistance="[0.01273  0.3864]/3"  Inductance="[0.9337e-3  4.1264e-3]/3"  Capacitance=[12.74e-9 7.751e-9]*3  Length=218  x1=[-0.00125 -1.55028860163576e-10 320589.458118059 -710064.570643251;-0.0012 -2.38681496354167e-10 333916.133277516 -703895.833049212;-0.00115 -3.22249330145613e-10 347124.169624802 -697477.004617374;-0.0011 -4.05702670284487e-10 360208.874407492 -690810.365926914;-0.00105 -4.8901186619641e-10 373165.598692283 -683898.285602815;-0.001 -5.72147318520761e-10 385989.73901673 -676743.219474304;-0.00095 -6.55079489627188e-10 398676.73902484 -669347.709702307;-0.0009 -7.3777891411019e-10 411222.091085921 -661714.383876231;-0.00085 -8.20216209258029e-10 423621.337896122 -653845.954080394;-0.0008 -9.02362085492275e-10 435870.074062091 -645745.215930437;-0.00075 -9.84187356774249e-10 447963.947666193 -637415.047580053;-0.0007 -1.06566295097469e-09 459898.661812722 -628858.40869839;-0.00065 -1.14675992020292e-09 471669.976154571 -620078.3394185;-0.0006 -1.22744945109194e-09 483273.708399804 -611077.959257191;-0.00055 -1.30770287503563e-09 494705.735797608 -601860.466006677;-0.0005 -1.38749167837461e-09 505961.996603083 -592429.134598422;-0.00045 -1.46678751252696e-09 517038.491520362 -582787.315939564;-0.0004 -1.54556220406039e-09 527931.285123544 -572938.435722364;-0.00035 -1.6237877647021e-09 538636.507254928 -562885.993207066;-0.0003 -1.70143640128287e-09 549150.354400067 -552633.559978629;-0.00025 -1.77848052561185e-09 559469.091039131 -542184.778677761;-0.0002 -1.85489276427853e-09 569589.050974127 -531543.361706707;-0.00015 -1.93064596837834e-09 579506.638631477 -520713.089910244;-0.0001 -2.0057132231586e-09 589218.330339511 -509697.811232373;-5e-05 -2.0800678575811e-09 598720.675580408 -498501.439349158]  x2=[-0.00125 1.52831318809478e-09 187223.160106197 -760871.621865356;-0.0012 1.40142405450867e-09 201531.158456881 -757207.601415491;-0.00115 1.27403700162903e-09 215767.553746581 -753274.548710377;-0.0011 1.1461972894692e-09 229927.287851837 -749073.861144911;-0.00105 1.01795033887017e-09 244005.329886545 -744607.031203385;-0.001 8.89341715362825e-10 257996.677989404 -739875.645929205;-0.00095 7.60417112978722e-10 271896.361101056 -734881.386361033;-0.0009 6.31222338015193e-10 285699.440730275 -729626.026935511;-0.00085 5.01803292760607e-10 299401.012708594 -724111.434856819;-0.0008 3.72205959185498e-10 312996.208932731 -718339.569433264;-0.00075 2.42476382605395e-10 326480.199094203 -712312.481381149;-0.0007 1.1266065532113e-10 339848.19239551 -706032.312096159;-0.00065 -1.71950997575227e-11 353095.439252287 -699501.292892537;-0.0006 -1.47044745499108e-10 366217.232980802 -692721.744210308;-0.00055 -2.76842146942788e-10 379208.911470227 -685696.074790838;-0.0005 -4.06541187689877e-10 392065.858839054 -678426.780821018;-0.00045 -5.36095786288772e-10 404783.507075103 -670916.44504638;-0.0004 -6.65459912607483e-10 417357.337658513 -663167.735853466;-0.00035 -7.94587604187911e-10 429782.883167149 -655183.406321755;-0.0003 -9.23432982576093e-10 442055.728863858 -646966.29324551;-0.00025 -1.0519502696226e-09 454171.514265002 -638519.316125882;-0.0002 -1.1800938037473e-09 466125.934689719 -629845.476133619;-0.00015 -1.30781805616268e-09 477914.742789354 -620947.85504277;-0.0001 -1.43507764705003e-09 489533.750056524 -611829.61413574;-5e-05 -1.56182736168268e-09 500978.828313271 -602493.993080107]  x3=[-0.00125 2.59683929486827e-11 221.284192839477 -3132.69922263436;-0.0012 2.58318116067639e-11 280.291443620253 -3127.97207788009;-0.00115 2.56860523451824e-11 339.199108185752 -3122.13357954075;-0.0011 2.55311669515098e-11 397.986256923249 -3115.18580200701;-0.00105 2.53672104557891e-11 456.632003038721 -3107.13121379114;-0.001 2.51942411109823e-11 515.115509977819 -3097.97267664998;-0.00095 2.50123203722742e-11 573.415998829006 -3087.71344456817;-0.0009 2.48215128752369e-11 631.512755706196 -3076.35716260202;-0.00085 2.46218864128657e-11 689.385139108307 -3063.90786558443;-0.0008 2.44135119114919e-11 747.012587253081 -3050.36997669136;-0.00075 2.41964634055838e-11 804.374625382593 -3035.74830587027;-0.0007 2.3970818011442e-11 861.450873037831 -3020.04804813118;-0.00065 2.37366558998007e-11 918.221051299779 -3003.2747817009;-0.0006 2.3494060267343e-11 974.664989994418 -2985.43446604113;-0.00055 2.32431173071421e-11 1030.76263485909 -2966.53343973107;-0.0005 2.29839161780368e-11 1086.4940546677 -2946.57841821538;-0.00045 2.27165489729541e-11 1141.83944831216 -2925.57649141817;-0.0004 2.24411106861888e-11 1196.77915183763 -2903.53512122404;-0.00035 2.21576991796527e-11 1251.29364542906 -2880.46213882687;-0.0003 2.18664151481046e-11 1305.36356034645 -2856.36574194743;-0.00025 2.15673620833738e-11 1358.9696858065 -2831.2544919208;-0.0002 2.12606462375904e-11 1412.09297580807 -2805.13731065454;-0.00015 2.09463765854339e-11 1464.71455589918 -2778.0234774588;-0.0001 2.06246647854151e-11 1516.81572988299 -2749.92262574941;-5e-05 2.0295625140205e-11 1568.37798646048 -2720.84473962517]  x4=[-0.00125 -1.16446607310931e-11 3048.851985329 -13840.8015991339;-0.0012 -1.22810678190566e-11 3309.1882137768 -13780.8767088441;-0.00115 -1.29131115021018e-11 3568.34870340934 -13716.055538679;-0.0011 -1.35405672181176e-11 3826.24137573867 -13646.3611192915;-0.00105 -1.41632120350758e-11 4082.7746027263 -13571.8182127771;-0.001 -1.47808247302378e-11 4337.85723933819 -13492.4533038756;-0.00095 -1.53931858687537e-11 4591.39865592817 -13408.294590561;-0.0009 -1.6000077881627e-11 4843.30877043818 -13319.3719740237;-0.00085 -1.66012851430151e-11 5093.49808040404 -13225.7170480457;-0.0008 -1.7196594046841e-11 5341.87769475523 -13127.3630877763;-0.00075 -1.77857930826856e-11 5588.35936539745 -13024.3450379094;-0.0007 -1.8368672910937e-11 5832.85551856678 -12916.6995002674;-0.00065 -1.89450264371679e-11 6075.27928594419 -12804.4647207974;-0.0006 -1.95146488857145e-11 6315.54453551946 -12687.6805759821;-0.00055 -2.00773378724334e-11 6553.56590219348 -12566.388558672;-0.0005 -2.06328934766068e-11 6789.25881810802 -12440.6317633433;-0.00045 -2.1181118311974e-11 7022.53954269234 -12310.4548707867;-0.0004 -2.17218175968613e-11 7253.3251924158 -12175.9041322322;-0.00035 -2.22547992233874e-11 7481.53377023596 -12037.0273529165;-0.0003 -2.27798738257183e-11 7707.08419473176 -11893.873875098;-0.00025 -2.3296854847348e-11 7929.89632891136 -11746.4945605258;-0.0002 -2.38055586073811e-11 8149.89100868443 -11594.9417723685;-0.00015 -2.43058043657941e-11 8366.99007098879 -11439.2693566102;-0.0001 -2.47974143876508e-11 8581.11638156134 -11279.532622919;-5e-05 -2.52802140062514e-11 8792.19386234351 -11115.7883249956]  x5=0.00123288061605072  V1=ones(3,3)  V2=ones(3,3)  I1=ones(3,3)  I2=ones(3,3)  nHarmo=1  Measurements=None
      settings: AttributesFormatString=\n  SourceProductName=Simscape Electrical
  LMO7 : powerlib/Measurements/Three-Phase V-I Measurement  VoltageMeasurement=no  SetLabelV=on  LabelV=Vabc_LMO7  Vpu=on  VpuLL=off  CurrentMeasurement=no  SetLabelI=off  LabelI=A1  Ipu=off  Pbase=100e6  Vbase=735e3  OutputType=Magnitude  PhasorSimulation=off  PSBequivalent=0
      settings: SourceProductName=Simscape Electrical
  LVD 990 Mvar : powerlib/Elements/Three-Phase Series RLC Load  LConnTagsString=A|B|C  Configuration=Y (grounded)  NominalVoltage=735e3  Vabc=[1e3 1e3 1e3]  Vabcp=[1e3 1e3 1e3]  NominalFrequency=60  UnbalancedPower=off  ActivePower=3300000  InductivePower=990e6  CapacitivePower=0  Pabc=[10e3 9e3 11e3]  QLabc=[100 90 110]  QCabc=[100 90 110]  Pabcp=[10e3 9e3 11e3]  QLabcp=[100 90 110]  QCabcp=[100 90 110]  Measurements=None  LoadType=constant Z
      settings: SourceProductName=Simscape Electrical
  LVD-MTL 3*260km : powerlib/Elements/Distributed Parameters Line  Phases=3  Frequency=60  Resistance="[0.01273  0.3864]/3"  Inductance="[0.9337e-3  4.1264e-3]/3"  Capacitance=[12.74e-9 7.751e-9]*3  Length=260  x1=[-0.0015 7.35594192207311e-09 -59599.4660795114 -791918.716753236;-0.00145 7.06449713285262e-09 -44662.4317893299 -792901.401182116;-0.0014 6.77054236143927e-09 -29709.5291497991 -793602.37151865;-0.00135 6.47418204856364e-09 -14746.0708560269 -794021.378711414;-0.0013 6.17552148963374e-09 222.626646505378 -794158.273889149;-0.00125 5.87466679732404e-09 15191.2450508502 -794013.008413649;-0.0012 5.57172486387417e-09 30154.4660781634 -793585.633897047;-0.00115 5.2668033231106e-09 45106.973367263 -792876.302183472;-0.0011 4.96001051220482e-09 60043.4543635075 -791885.265295106;-0.00105 4.65145543318174e-09 74958.6022063205 -790612.875342636;-0.001 4.3412477141917e-09 89847.1176146939 -789059.584400153;-0.00095 4.02949757056018e-09 104703.710769997 -787225.944344533;-0.0009 3.71631576562876e-09 119523.103195422 -785112.606659357;-0.00085 3.40181357140148e-09 134300.029631405 -782720.32220344;-0.0008 3.08610272901043e-09 149029.239906345 -780049.94094406;-0.00075 2.76929540901461e-09 163705.500801967 -777102.411654963;-0.0007 2.45150417154628e-09 178323.597912657 -773878.781579269;-0.00065 2.13284192631893e-09 192878.337498118 -770380.196057396;-0.0006 1.81342189251094e-09 207364.548328679 -766607.898120119;-0.00055 1.49335755853937e-09 221777.083522609 -762563.228046935;-0.0005 1.17276264173804e-09 236110.822374781 -758247.62288986;-0.00045 8.51751047954349e-10 250360.672176033 -753662.615962858;-0.0004 5.30436831079034e-10 264521.570022583 -748809.836297057;-0.00035 2.08934152523375e-10 278588.484614854 -743691.008061967;-0.0003 -1.12642759341812e-10 292556.418045074 -738307.949952885;-0.00025 -4.34179649770966e-10 306420.407573005 -732662.574544725;-0.0002 -7.55562278237954e-10 320175.527389181 -726756.887612489;-0.00015 -1.07667645902518e-09 333816.89036503 -720592.987418623;-0.0001 -1.39740810179324e-09 347339.64978924 -714173.063967515;-5e-05 -1.71764325211666e-09 360739.00108978 -707499.398227399]  x2=[-0.0015 1.06223134218054e-08 -301447.229390913 -704347.974560849;-0.00145 1.01718498464045e-08 -288117.810949931 -709904.664194201;-0.0014 9.71777226118765e-09 -274686.025622627 -715209.12808066;-0.00135 9.26024199775871e-09 -261156.645658368 -720259.481569465;-0.0013 8.79942161444169e-09 -247534.477981436 -725053.930294069;-0.00125 8.33547483852455e-09 -233824.362483141 -729590.770809669;-0.0012 7.86856650808763e-09 -220031.170302238 -733868.391198433;-0.00115 7.39886251343749e-09 -206159.802094231 -737885.271642205;-0.0011 6.92652973816689e-09 -192215.186290195 -741639.98496249;-0.00105 6.4517359998618e-09 -178202.277345724 -745131.197127525;-0.001 5.97464999047667e-09 -164126.053980644 -748357.66772625;-0.00095 5.49544121639892e-09 -149991.517410091 -751318.250409025;-0.0009 5.01427993822417e-09 -135803.689567603 -754011.893294921;-0.00085 4.53133711026346e-09 -121567.611320858 -756437.639345445;-0.0008 4.04678431980397e-09 -107288.340680669 -758594.626704578;-0.00075 3.5607937261449e-09 -92970.9510039021 -760482.08900498;-0.0007 3.07353799943006e-09 -78620.5291909357 -762099.355640283;-0.00065 2.58519025929904e-09 -64242.1738783088 -763445.852003354;-0.0006 2.09592401337858e-09 -49840.9936271995 -764521.099690445;-0.00055 1.60591309563616e-09 -35422.1051083783 -765324.716671174;-0.0005 1.1153316046176e-09 -20990.6312842786 -765856.417424254;-0.00045 6.24353841590709e-10 -6551.69958883295 -766116.013038938;-0.0004 1.33154248616831e-10 7889.55989427991 -766103.411282142;-0.00035 -3.58092653427551e-10 22328.0162543294 -765818.616631209;-0.0003 -8.49212326857271e-10 36758.5395765212 -765261.730272322;-0.00025 -1.34003027919088e-09 51176.0027646316 -764432.950064554;-0.0002 -1.83037212514701e-09 65575.2833626403 -763332.570469565;-0.00015 -2.32006364860261e-09 79951.2653747147 -761960.982446987;-0.0001 -2.80893086449111e-09 94298.8410828989 -760318.673315513;-5e-05 -3.29680008061852e-09 108612.912861861 -758406.226579756]  x3=[-0.0015 1.06625757187899e-10 478.440094937282 -458.994464498088;-0.00145 1.05847264458705e-10 487.006448674426 -449.895407456498;-0.0014 1.05031164700453e-10 495.399771339294 -440.636504718868;-0.00135 1.04177747869502e-10 503.61708082431 -431.221045929255;-0.0013 1.03287317180787e-10 511.655457558541 -421.652376355333;-0.00125 1.02360189000092e-10 519.512045545009 -411.933895699839;-0.0012 1.01396692731646e-10 527.184053375413 -402.069056892675;-0.00115 1.00397170701085e-10 534.668755221902 -392.061364864096;-0.0011 9.93619780338261e-11 541.963491805549 -381.914375299428;-0.00105 9.8291482528896e-11 549.06567134118 -371.631693375746;-0.001 9.71860645282498e-11 555.972770458225 -361.216972480975;-0.00095 9.60461167816397e-11 562.682335097256 -350.67391291586;-0.0009 9.4872044307072e-11 569.191981381906 -340.006260579261;-0.00085 9.36642642469064e-11 575.499396465845 -329.217805637257;-0.0008 9.24232057196473e-11 581.602339354528 -318.312381176521;-0.00075 9.114930966748e-11 587.498641701407 -307.293861842434;-0.0007 8.98430286996061e-11 593.186208578333 -296.166162462451;-0.00065 8.85048269314334e-11 598.663019219878 -284.933236655175;-0.0006 8.71351798196781e-11 603.927127741298 -273.599075425659;-0.00055 8.57345739934374e-11 608.976663829902 -262.167705747418;-0.0005 8.4303507081292e-11 613.809833409562 -250.643189131667;-0.00045 8.28424875345018e-11 618.424919278139 -239.029620184285;-0.0004 8.13520344463549e-11 622.8202817176 -227.33112515102;-0.00035 7.98326773677364e-11 626.994359076599 -215.551860451452;-0.0003 7.8284956118982e-11 630.945668325326 -203.696011202242;-0.00025 7.67094205980815e-11 634.672805582419 -191.767789730174;-0.0002 7.51066305853035e-11 638.174446613758 -179.771434075539;-0.00015 7.34771555443076e-11 641.449347302958 -167.711206486381;-0.0001 7.18215744198169e-11 644.496344093398 -155.591391904135;-5e-05 7.01404754319218e-11 647.314354401627 -143.416296441212]  x4=[-0.0015 2.25577725789584e-12 -7254.99969893002 -15290.6542920098;-0.00145 5.45888317046172e-13 -6965.50564706586 -15424.6831660543;-0.0014 -1.16419457532322e-12 -6673.53678421237 -15553.2317236163;-0.00135 -2.87386383490344e-12 -6379.19684551629 -15676.2542920055;-0.0013 -4.58251202434737e-12 -6082.59040855629 -15793.7071618891;-0.00125 -6.28953206908922e-12 -5783.8228561871 -15905.5486028217;-0.0012 -7.99431747303527e-12 -5483.00033909746 -16011.7388780718;-0.00115 -9.69626253404905e-12 -5180.2297380953 -16112.2402587403;-0.0011 -1.13947625591544e-11 -4875.61862613347 -16207.0170371653;-0.00105 -1.30892140793799e-11 -4569.2752300896 -16296.0355396085;-0.001 -1.47790150641689e-11 -4261.30839231363 -16379.26413822;-0.00095 -1.64635651352776e-11 -3951.82753195659 -16456.6732622751;-0.0009 -1.8142265780087e-11 -3640.94260609454 -16528.2354086804;-0.00085 -1.98145205642512e-11 -3328.76407066132 -16593.9251517461;-0.0008 -2.14797353436082e-11 -3015.40284120411 -16653.7191522194;-0.00075 -2.31373184752758e-11 -2700.9702534756 -16707.5961655766;-0.0007 -2.47866810278603e-11 -2385.57802387703 -16755.5370495713;-0.00065 -2.64272369907002e-11 -2069.33820976578 -16797.5247710357;-0.0006 -2.80584034820738e-11 -1752.363169642 -16833.5444119324;-0.00055 -2.96796009562936e-11 -1434.76552322813 -16863.5831746545;-0.0005 -3.12902534096165e-11 -1116.65811145567 -16887.6303865725;-0.00045 -3.28897885848953e-11 -798.153956373301 -16905.6775038267;-0.0004 -3.44776381748984e-11 -479.36622099074 -16917.7181143621;-0.00035 -3.60532380242274e-11 -160.408169072418 -16923.7479402071;-0.0003 -3.7616028329758e-11 158.606875104572 -16923.7648389935;-0.00025 -3.91654538395363e-11 477.565567014062 -16917.7688047171;-0.0002 -4.07009640500563e-11 796.354582151578 -16905.7619677403;-0.00015 -4.22220134018518e-11 1114.86065629799 -16887.7485940351;-0.0001 -4.37280614733307e-11 1432.97062576176 -16863.7350836675;-5e-05 -4.52185731727845e-11 1750.57146758546 -16833.7299685233]  x5=0.00147040807418893  V1=ones(3,3)  V2=ones(3,3)  I1=ones(3,3)  I2=ones(3,3)  nHarmo=1  Measurements=None
      settings: AttributesFormatString=\n  SourceProductName=Simscape Electrical
  LVD7 : powerlib/Measurements/Three-Phase V-I Measurement  VoltageMeasurement=no  SetLabelV=on  LabelV=Vabc_LVD7  Vpu=on  VpuLL=off  CurrentMeasurement=no  SetLabelI=off  LabelI=A1  Ipu=off  Pbase=100e6  Vbase=735e3  OutputType=Magnitude  PhasorSimulation=off  PSBequivalent=0
      settings: SourceProductName=Simscape Electrical
  Load Flow Bus1 : powerlib/Measurements/Load Flow Bus  LConnTagsString=a  Phases=single  Connectors=on one side  ID=LG31_13.8  Vbase=13.8e3  Vref=1  Vangle=0  VLF=1  VLFb=1  VLFc=1  angleLF=0.615  angleLFb=0  angleLFc=0
      settings: AttributesFormatString=%<ID>\n%<Vbase>V\n%<VLF>pu\n%<angleLF>deg.  SourceProductName=Simscape Electrical
  Load Flow Bus10 : powerlib/Measurements/Load Flow Bus  LConnTagsString=a  Phases=single  Connectors=on one side  ID=LVD7  Vbase=735e3  Vref=1  Vangle=0  VLF=1.077  VLFb=1  VLFc=1  angleLF=-8.632  angleLFb=0  angleLFc=0
      settings: AttributesFormatString=%<ID>\n%<Vbase>V\n%<VLF>pu\n%<angleLF>deg.  SourceProductName=Simscape Electrical
  Load Flow Bus11 : powerlib/Measurements/Load Flow Bus  LConnTagsString=a  Phases=single  Connectors=on one side  ID=CHM7  Vbase=735e3  Vref=1  Vangle=0  VLF=1.07  VLFb=1  VLFc=1  angleLF=-1.497  angleLFb=0  angleLFc=0
      settings: AttributesFormatString=%<ID>\n%<Vbase>V\n%<VLF>pu\n%<angleLF>deg.  SourceProductName=Simscape Electrical
  Load Flow Bus12 : powerlib/Measurements/Load Flow Bus  LConnTagsString=a  Phases=single  Connectors=on one side  ID=LG47  Vbase=735e3  Vref=1  Vangle=0  VLF=1.012  VLFb=1  VLFc=1  angleLF=21.74  angleLFb=0  angleLFc=0
      settings: AttributesFormatString=%<ID>\n%<Vbase>V\n%<VLF>pu\n%<angleLF>deg.  SourceProductName=Simscape Electrical
  Load Flow Bus2 : powerlib/Measurements/Load Flow Bus  LConnTagsString=a  Phases=single  Connectors=on one side  ID=LG3_13.8  Vbase=13.8e3  Vref=1  Vangle=0  VLF=1  VLFb=1  VLFc=1  angleLF=0.05131  angleLFb=0  angleLFc=0
      settings: AttributesFormatString=%<ID>\n%<Vbase>V\n%<VLF>pu\n%<angleLF>deg.  SourceProductName=Simscape Electrical
  Load Flow Bus3 : powerlib/Measurements/Load Flow Bus  LConnTagsString=a  Phases=single  Connectors=on one side  ID=LG4_13.8  Vbase=13.8e3  Vref=1  Vangle=0  VLF=1  VLFb=1  VLFc=1  angleLF=-2.292  angleLFb=0  angleLFc=0
      settings: AttributesFormatString=%<ID>\n%<Vbase>V\n%<VLF>pu\n%<angleLF>deg.  SourceProductName=Simscape Electrical
  Load Flow Bus4 : powerlib/Measurements/Load Flow Bus  LConnTagsString=a  Phases=single  Connectors=on one side  ID=LG2_13.8  Vbase=13.8e3  Vref=1  Vangle=0  VLF=1  VLFb=1  VLFc=1  angleLF=0  angleLFb=0  angleLFc=0
      settings: AttributesFormatString=%<ID>\n%<Vbase>V\n%<VLF>pu\n%<angleLF>deg.  SourceProductName=Simscape Electrical
  Load Flow Bus5 : powerlib/Measurements/Load Flow Bus  LConnTagsString=a  Phases=single  Connectors=on one side  ID=LG27  Vbase=735e3  Vref=1  Vangle=0  VLF=1.008  VLFb=1  VLFc=1  angleLF=23.79  angleLFb=0  angleLFc=0
      settings: AttributesFormatString=%<ID>\n%<Vbase>V\n%<VLF>pu\n%<angleLF>deg.  SourceProductName=Simscape Electrical
  Load Flow Bus6 : powerlib/Measurements/Load Flow Bus  LConnTagsString=a  Phases=single  Connectors=on one side  ID=LG37  Vbase=735e3  Vref=1  Vangle=0  VLF=1  VLFb=1  VLFc=1  angleLF=24.78  angleLFb=0  angleLFc=0
      settings: AttributesFormatString=%<ID>\n%<Vbase>V\n%<VLF>pu\n%<angleLF>deg.  SourceProductName=Simscape Electrical
  Load Flow Bus7 : powerlib/Measurements/Load Flow Bus  LConnTagsString=a  Phases=single  Connectors=on one side  ID=LMO7  Vbase=735e3  Vref=1  Vangle=0  VLF=1.029  VLFb=1  VLFc=1  angleLF=18.4  angleLFb=0  angleLFc=0
      settings: AttributesFormatString=%<ID>\n%<Vbase>V\n%<VLF>pu\n%<angleLF>deg.  SourceProductName=Simscape Electrical
  Load Flow Bus8 : powerlib/Measurements/Load Flow Bus  LConnTagsString=a  Phases=single  Connectors=on one side  ID=NEM_ALB7  Vbase=735e3  Vref=1  Vangle=0  VLF=1.049  VLFb=1  VLFc=1  angleLF=10.43  angleLFb=0  angleLFc=0
      settings: AttributesFormatString=%<ID>\n%<Vbase>V\n%<VLF>pu\n%<angleLF>deg.  SourceProductName=Simscape Electrical
  Load Flow Bus9 : powerlib/Measurements/Load Flow Bus  LConnTagsString=a  Phases=single  Connectors=on one side  ID=ABI_CHB7  Vbase=735e3  Vref=1  Vangle=0  VLF=1.071  VLFb=1  VLFc=1  angleLF=2.371  angleLFb=0  angleLFc=0
      settings: AttributesFormatString=%<ID>\n%<Vbase>V\n%<VLF>pu\n%<angleLF>deg.  SourceProductName=Simscape Electrical
  NEM-ABI 6*236 : powerlib/Elements/Distributed Parameters Line  Phases=3  Frequency=60  Resistance="[0.01273  0.3864]/6"  Inductance="[0.9337e-3  4.1264e-3]/6"  Capacitance=[12.74e-9 7.751e-9]*6  Length=236  x1=[-0.00135 1.95298291285449e-09 0 0;-0.0013 1.8258679735382e-09 0 0;-0.00125 1.69810431202501e-09 0 0;-0.0012 1.56973732213547e-09 0 0;-0.00115 1.44081261204987e-09 0 0;-0.0011 1.31137598810381e-09 0 0;-0.00105 1.18147343851344e-09 0 0;-0.001 1.0511511170361e-09 0 0;-0.00095 9.20455326572057e-10 0 0;-0.0009 7.89432502713336e-10 0 0;-0.00085 6.58129197245378e-10 327613.765821609 -714456.409844664;-0.0008 5.26592061607399e-10 341021.968478473 -708154.494226726;-0.00075 3.94867830317361e-10 354309.007653752 -701600.97468895;-0.0007 2.6300330436742e-10 367470.162525697 -694798.179665623;-0.00065 1.3104533459576e-10 380500.756998648 -687748.526157425;-0.0006 -9.59194959295059e-13 393396.161364438 -680454.518872678;-0.00055 -1.32963383716948e-10 406151.793947297 -672918.749337441;-0.0005 -2.64920331217487e-10 418763.122731706 -665143.894974746;-0.00045 -3.96783153785794e-10 431225.666972598 -657132.718153328;-0.0004 -5.28505001188891e-10 443534.998787347 -648888.065206164;-0.00035 -6.60039073281604e-10 455686.744728971 -640412.86541919;-0.0003 -7.91338636634435e-10 467676.587339999 -631710.129990535;-0.00025 -9.22357041137721e-10 479500.266686443 -622782.950960655;-0.0002 -1.0530477365762e-09 491153.58187133 -613634.500113755;-0.00015 -1.18336428916809e-09 502632.392527263 -604268.027850856;-0.0001 -1.31326039806277e-09 513932.620287475 -594686.862034956;-5e-05 -1.44268991179125e-09 525050.25023485 -584894.406808647]  x2=[-0.00135 2.26927582972027e-09 0 0;-0.0013 2.07287685060179e-09 0 0;-0.00125 1.87574138820853e-09 0 0;-0.0012 1.67793948383161e-09 0 0;-0.00115 1.47954141554579e-09 0 0;-0.0011 1.28061767324004e-09 0 0;-0.00105 1.0812389335728e-09 0 0;-0.001 8.81476034860901e-10 0 0;-0.00095 6.81399951911074e-10 0 0;-0.0009 4.81081770802897e-10 0 0;-0.00085 2.80592663632282e-10 157243.615145399 -773711.427173535;-0.0008 8.00038632243545e-11 171798.947031464 -770610.196625785;-0.00075 -1.2061336217523e-10 186293.239569689 -767235.171944525;-0.0007 -3.21187734221548e-10 200721.343006953 -763587.552259953;-0.00065 -5.2164798979527e-10 215078.131106804 -759668.633553976;-0.0006 -7.21922906322107e-10 229358.502970793 -755479.808199749;-0.00055 -9.21941327077848e-10 243557.384850794 -751022.564466975;-0.0005 -1.12163218647001e-09 257669.731951685 -746298.485993128;-0.00045 -1.32092453528711e-09 271690.530223738 -741309.251220797;-0.0004 -1.51974756590655e-09 285614.79814409 -736056.632801338;-0.00035 -1.71803063745229e-09 299437.588486649 -730542.496965065;-0.0003 -1.91570330089314e-09 313153.990079826 -724768.802858185;-0.00025 -2.11269532407304e-09 326759.129551448 -718737.601846722;-0.0002 -2.30893671666413e-09 340248.173060242 -712451.036787676;-0.00015 -2.50435775503408e-09 353616.32801328 -705911.341267679;-0.0001 -2.69888900701845e-09 366858.84476876 -699120.83880941;-5e-05 -2.89246135658971e-09 379971.018323536 -692081.942046059]  x3=[-0.00135 7.96200460911348e-11 0 0;-0.0013 7.85853243566919e-11 0 0;-0.00125 7.75226816306984e-11 0 0;-0.0012 7.64324954650549e-11 0 0;-0.00115 7.5315153197715e-11 0 0;-0.0011 7.41710518150659e-11 0 0;-0.00105 7.30005978108812e-11 0 0;-0.001 7.18042070418952e-11 0 0;-0.00095 7.05823045800515e-11 0 0;-0.0009 6.93353245614764e-11 0 0;-0.00085 6.80637100322329e-11 6.88825081738219 -4556.57125523285;-0.0008 6.67679127909084e-11 92.7716411794549 -4555.63231352019;-0.00075 6.54483932280926e-11 178.62207021916 -4553.07477733871;-0.0007 6.41056201628031e-11 264.409035687847 -4548.89955536885;-0.00065 6.27400706759162e-11 350.102057885167 -4543.10813104708;-0.0006 6.13522299406625e-11 435.670690488374 -4535.7025620389;-0.00055 5.99425910502467e-11 521.084531369748 -4526.68547950772;-0.0005 5.85116548426544e-11 606.313233398332 -4516.06008718001;-0.00045 5.70599297227067e-11 691.326515222121 -4503.83016020707;-0.0004 5.55879314814262e-11 776.094172026884 -4490.00004382374;-0.00035 5.40961831127787e-11 860.586086267791 -4474.5746518045;-0.0003 5.25852146278567e-11 944.772238370028 -4457.55946471769;-0.00025 5.10555628665681e-11 1028.62271739462 -4438.96052797826;-0.0002 4.95077713069001e-11 1112.10773166563 -4418.78444969987;-0.00015 4.79423898718238e-11 1195.197619355 -4397.03839834707;-0.0001 4.63599747339094e-11 1277.8628590213 -4373.73010018836;-5e-05 4.47610881177206e-11 1360.07408009848 -4348.86783655107]  x4=[-0.00135 -1.23974386905571e-11 0 0;-0.0013 -1.37611595791231e-11 0 0;-0.00125 -1.51199911932161e-11 0 0;-0.0012 -1.64734507464337e-11 0 0;-0.00115 -1.78210573610414e-11 0 0;-0.0011 -1.91623322388258e-11 0 0;-0.00105 -2.04967988312094e-11 0 0;-0.001 -2.18239830085662e-11 0 0;-0.00095 -2.31434132286776e-11 0 0;-0.0009 -2.44546207042689e-11 0 0;-0.00085 -2.57571395695675e-11 5577.08620259223 -29803.1318203087;-0.0008 -2.70505070458228e-11 6137.8383046953 -29692.7181709472;-0.00075 -2.83342636057288e-11 6696.40966207476 -29571.7548402049;-0.0007 -2.96079531366926e-11 7252.60181698703 -29440.2848057773;-0.00065 -3.08711231028888e-11 7806.21715700783 -29298.3547783416;-0.0006 -3.2123324706043e-11 8357.05898524298 -29146.0151849607;-0.00055 -3.33641130448881e-11 8904.9315902138 -28983.3201511668;-0.0005 -3.45930472732356e-11 9449.64031539249 -28810.3274817307;-0.00045 -3.58096907566057e-11 9990.9916283627 -28627.0986401241;-0.0004 -3.70136112273621e-11 10528.7931895806 -28433.698726682;-0.00035 -3.82043809382941e-11 11062.8539207124 -28230.1964554727;-0.0003 -3.93815768145934e-11 11592.9840725233 -28016.6641298841;-0.00025 -4.05447806041704e-11 12118.9952922945 -27793.1776169349;-0.0002 -4.16935790262576e-11 12640.7006907444 -27559.8163203189;-0.00015 -4.28275639182457e-11 13157.914908429 -27316.6631521936;-0.0001 -4.39463323807021e-11 13670.4541815997 -27063.8045037218;-5e-05 -4.50494869205192e-11 14178.1364074931 -26801.3302143774]  x5=0.00133467809810995  V1=ones(3,3)  V2=ones(3,3)  I1=ones(3,3)  I2=ones(3,3)  nHarmo=1  Measurements=None
      settings: AttributesFormatString=\n  SourceProductName=Simscape Electrical
  NEM-ALB 1980 Mvar : powerlib/Elements/Three-Phase Series RLC Load  LConnTagsString=A|B|C  Configuration=Y (grounded)  NominalVoltage=735e3  Vabc=[1e3 1e3 1e3]  Vabcp=[1e3 1e3 1e3]  NominalFrequency=60  UnbalancedPower=off  ActivePower=6600000  InductivePower=1980e6  CapacitivePower=0  Pabc=[10e3 9e3 11e3]  QLabc=[100 90 110]  QCabc=[100 90 110]  Pabcp=[10e3 9e3 11e3]  QLabcp=[100 90 110]  QCabcp=[100 90 110]  Measurements=None  LoadType=constant Z
      settings: SourceProductName=Simscape Electrical
  NEM-ALB7 : powerlib/Measurements/Three-Phase V-I Measurement  VoltageMeasurement=no  SetLabelV=on  LabelV=Vabc_NEM7  Vpu=on  VpuLL=off  CurrentMeasurement=no  SetLabelI=off  LabelI=A1  Ipu=off  Pbase=100e6  Vbase=735e3  OutputType=Magnitude  PhasorSimulation=off  PSBequivalent=0
      settings: SourceProductName=Simscape Electrical
  Regulators1 : Subsystem
  Regulators2 : Subsystem
  Regulators3 : Subsystem
  Regulators4 : Subsystem
  MTLa : PMIOPort  Side=Right
  MTLb : PMIOPort  Port=2  Side=Right
  MTLc : PMIOPort  Port=3  Side=Right
  CHM7a : PMIOPort  Port=4  Side=Right
  CHM7b : PMIOPort  Port=5  Side=Right
  CHM7c : PMIOPort  Port=6  Side=Right
  wires:
  Regulators2/1(Pm) -> LG3_2200 MVA/1
  Regulators4/2(Vf) -> LG4-2700 MVA/2
  Regulators4/1(Pm) -> LG4-2700 MVA/1
  Regulators3/2(Vf) -> LG31-200 MVA/2
  Regulators3/1(Pm) -> LG31-200 MVA/1
  Regulators2/2(Vf) -> LG3_2200 MVA/2
  LG3_2200 MVA/1 -> Regulators2/1(m)
  Regulators1/1(Pm) -> LG2_6375 MVA/1
  Regulators1/2(Vf) -> LG2_6375 MVA/2
  LG2_6375 MVA/1 -> Regulators1/1(m)
  LG31-200 MVA/1 -> Regulators3/1(m)
  LG4-2700 MVA/1 -> Regulators4/1(m)
  connections:
  LG2-NENI 3*279km/RConn1 -- "Cs NEM "/LConn1
  LG2-NENI 3*279km/RConn2 -- "Cs NEM "/LConn2
  LG2-NENI 3*279km/RConn3 -- "Cs NEM "/LConn3
  CHB-CHM 3*195km/RConn1 -- "Cs  CHMN "/LConn1
  CHB-CHM 3*195km/RConn2 -- "Cs  CHMN "/LConn2
  CHB-CHM 3*195km/RConn3 -- "Cs  CHMN "/LConn3
  Load Flow Bus2/LConn1 -- 2200 MVA 13.8 kV/735 kV/LConn1 -- LG3_2200 MVA/RConn1 -- 110 MW/LConn1
  2200 MVA 13.8 kV/735 kV/LConn2 -- LG3_2200 MVA/RConn2 -- 110 MW/LConn2
  2200 MVA 13.8 kV/735 kV/LConn3 -- LG3_2200 MVA/RConn3 -- 110 MW/LConn3
  Load Flow Bus1/LConn1 -- 200 MVA 13.8 kV/735 kV/LConn1 -- LG31-200 MVA/RConn1 -- 10 MW/LConn1
  200 MVA 13.8 kV/735 kV/LConn2 -- LG31-200 MVA/RConn2 -- 10 MW/LConn2
  200 MVA 13.8 kV/735 kV/LConn3 -- LG31-200 MVA/RConn3 -- 10 MW/LConn3
  Load Flow Bus6/LConn1 -- 2200 MVA 13.8 kV/735 kV/RConn1 -- 200 MVA 13.8 kV/735 kV/RConn1 -- LG3-LMO 104km/LConn1 -- LG3 660 Mvar/LConn1 -- LG2-LG3 155km/RConn1
  2200 MVA 13.8 kV/735 kV/RConn2 -- LG3 660 Mvar/LConn2 -- LG2-LG3 155km/RConn2 -- 200 MVA 13.8 kV/735 kV/RConn2 -- LG3-LMO 104km/LConn2
  LG3-LMO 104km/RConn1 -- LMO7/RConn1 -- LG4-LMO 3*118km/RConn1 -- LMO 330 Mvar/LConn1
  LG3-LMO 104km/RConn2 -- LMO7/RConn2 -- LG4-LMO 3*118km/RConn2 -- LMO 330 Mvar/LConn2
  LG3-LMO 104km/RConn3 -- LMO7/RConn3 -- LG4-LMO 3*118km/RConn3 -- LMO 330 Mvar/LConn3
  LG4-LMO 3*118km/LConn1 -- LG4 660 Mvar/LConn1 -- 2700 MVA 13.8 kV/735 kV/RConn1 -- Load Flow Bus12/LConn1
  LG4-LMO 3*118km/LConn2 -- 2700 MVA 13.8 kV/735 kV/RConn2 -- LG4 660 Mvar/LConn2
  LG4 660 Mvar/LConn3 -- 2700 MVA 13.8 kV/735 kV/RConn3 -- LG4-LMO 3*118km/LConn3
  Load Flow Bus3/LConn1 -- LG4-2700 MVA/RConn1 -- 2700 MVA 13.8 kV/735 kV/LConn1 -- 135 MW/LConn1
  LG4-2700 MVA/RConn2 -- 2700 MVA 13.8 kV/735 kV/LConn2 -- 135 MW/LConn2
  LG4-2700 MVA/RConn3 -- 2700 MVA 13.8 kV/735 kV/LConn3 -- 135 MW/LConn3
  Load Flow Bus4/LConn1 -- 6375 MVA 13.8 kV/735 kV/LConn1 -- LG2_6375 MVA/RConn1 -- 275 MW/LConn1
  LG2_6375 MVA/RConn2 -- 6375 MVA 13.8 kV/735 kV/LConn2 -- 275 MW/LConn2
  LG2_6375 MVA/RConn3 -- 6375 MVA 13.8 kV/735 kV/LConn3 -- 275 MW/LConn3
  6375 MVA 13.8 kV/735 kV/RConn1 -- LG2-NENI 3*279km/LConn1 -- Load Flow Bus5/LConn1 -- LG2 660 Mvar/LConn1 -- LG2-LG3 155km/LConn1 -- LG27_nodes/LConn1
  6375 MVA 13.8 kV/735 kV/RConn2 -- LG2-NENI 3*279km/LConn2 -- LG2 660 Mvar/LConn2 -- LG2-LG3 155km/LConn2 -- LG27_nodes/LConn2
  6375 MVA 13.8 kV/735 kV/RConn3 -- LG2-NENI 3*279km/LConn3 -- LG2 660 Mvar/LConn3 -- LG27_nodes/LConn3 -- LG2-LG3 155km/LConn3
  "Cs NEM "/RConn1 -- NEM-ALB7/LConn1 -- Cs ALB/RConn1
  "Cs NEM "/RConn2 -- NEM-ALB7/LConn2 -- Cs ALB/RConn2
  "Cs NEM "/RConn3 -- NEM-ALB7/LConn3 -- Cs ALB/RConn3
  LMO7/LConn1 -- LMO-ALB 3*218km/LConn1
  LMO7/LConn2 -- LMO-ALB 3*218km/LConn2
  Load Flow Bus7/LConn1 -- LMO7/LConn3 -- LMO-ALB 3*218km/LConn3
  Cs ALB/LConn1 -- LMO-ALB 3*218km/RConn1
  Cs ALB/LConn2 -- LMO-ALB 3*218km/RConn2
  Cs ALB/LConn3 -- LMO-ALB 3*218km/RConn3
  200 MVA 13.8 kV/735 kV/RConn3 -- LG3-LMO 104km/LConn3 -- LG3 660 Mvar/LConn3 -- LG2-LG3 155km/RConn3 -- 2200 MVA 13.8 kV/735 kV/RConn3
  Load Flow Bus8/LConn1 -- NEM-ABI 6*236/LConn1 -- NEM-ALB7/RConn1 -- NEM-ALB 1980 Mvar/LConn1
  NEM-ALB 1980 Mvar/LConn2 -- NEM-ALB7/RConn2 -- NEM-ABI 6*236/LConn2
  NEM-ALB 1980 Mvar/LConn3 -- NEM-ALB7/RConn3 -- NEM-ABI 6*236/LConn3
  NEM-ABI 6*236/RConn1 -- "Cs ABI+CHB "/LConn1
  NEM-ABI 6*236/RConn2 -- "Cs ABI+CHB "/LConn2
  NEM-ABI 6*236/RConn3 -- "Cs ABI+CHB "/LConn3
  "Cs ABI+CHB "/RConn1 -- ABI-CHB7/LConn1
  "Cs ABI+CHB "/RConn2 -- ABI-CHB7/LConn2
  "Cs ABI+CHB "/RConn3 -- ABI-CHB7/LConn3
  Load Flow Bus9/LConn1 -- ABI+CHB 1320 Mvar/LConn1 -- CHB-CHM 3*195km/LConn1 -- ABI-CHB 3*271km/LConn1 -- ABI-CHB7/RConn1
  ABI-CHB 3*271km/LConn2 -- ABI-CHB7/RConn2 -- ABI+CHB 1320 Mvar/LConn2 -- CHB-CHM 3*195km/LConn2
  ABI-CHB 3*271km/LConn3 -- ABI-CHB7/RConn3 -- ABI+CHB 1320 Mvar/LConn3 -- CHB-CHM 3*195km/LConn3
  ABI-CHB 3*271km/RConn1 -- "Cs LVDN "/LConn1
  ABI-CHB 3*271km/RConn2 -- "Cs LVDN "/LConn2
  ABI-CHB 3*271km/RConn3 -- "Cs LVDN "/LConn3
  "Cs LVDN "/RConn1 -- LVD7/LConn1
  "Cs LVDN "/RConn2 -- LVD7/LConn2
  "Cs LVDN "/RConn3 -- LVD7/LConn3
  "Cs LVDS "/LConn1 -- LVD 990 Mvar/LConn1 -- Load Flow Bus10/LConn1 -- LVD7/RConn1
  "Cs LVDS "/LConn2 -- LVD7/RConn2 -- LVD 990 Mvar/LConn2
  "Cs LVDS "/LConn3 -- LVD7/RConn3 -- LVD 990 Mvar/LConn3
  "Cs LVDS "/RConn1 -- LVD-MTL 3*260km/LConn1
  "Cs LVDS "/RConn2 -- LVD-MTL 3*260km/LConn2
  "Cs LVDS "/RConn3 -- LVD-MTL 3*260km/LConn3
  MTLa/RConn1 -- LVD-MTL 3*260km/RConn1
  MTLb/RConn1 -- LVD-MTL 3*260km/RConn2
  MTLc/RConn1 -- LVD-MTL 3*260km/RConn3
  "Cs  CHMN "/RConn1 -- CHM7/LConn1
  "Cs  CHMN "/RConn2 -- CHM7/LConn2
  "Cs  CHMN "/RConn3 -- CHM7/LConn3
  CHM 1320Mvar/LConn2 -- CHM7/RConn2 -- CHM7b/RConn1
  Load Flow Bus11/LConn1 -- CHM 1320Mvar/LConn3 -- CHM7c/RConn1 -- CHM7/RConn3
  CHM7a/RConn1 -- CHM 1320Mvar/LConn1 -- CHM7/RConn1
